simulink model "three_a_attitude_control_euler"  (R2021a)
settings: Solver=ode23t  StartTime=0.0  StopTime=100  RelTol=1e-5
undefined symbols (not defined in the file): eul_0, eul_init, g, I, km, kt, L, m, pm_0, sigbuilder_block, thrust_max, TQ_max_per_motor, Vb_init, Vm_0, wb_init, Xe_init, xme_0
libraries: simulink_extras x15, pid_lib x5, simulink x1
(part 1 of 2)
settings Model: Creator=Petronas-Tareq  LastModifiedBy=Petronas-Tareq

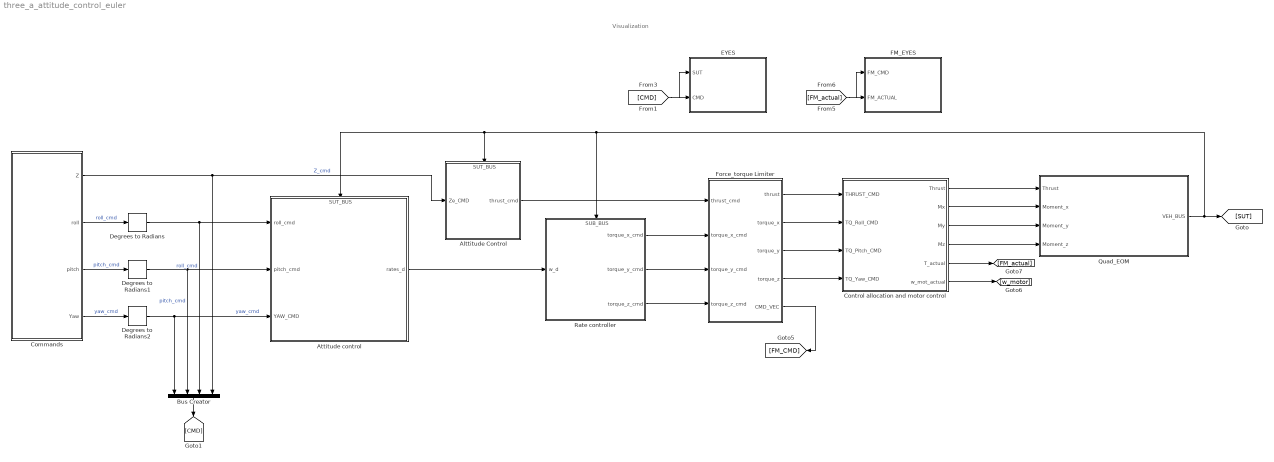
== system three_a_attitude_control_euler ==
  note: Visualization
  Alttitude Control : Subsystem
      settings: PortSchema="{\"entries\":[{\"content\":{\"sides\":[{\"content\":{\"connectorIds\":[\"In1\"]},\"type\":\"ConnectorPlacement.EquallySpacedRectSide\",\"uuid\":\"04a4dd9c-9e09-4d9f-8b40-74299d59d50a\"},{\"content\":{\"connectorIds\":[\"Out1\"],\"side\":\"RIGHT\"},\"type\":\"ConnectorPlacement.EquallySpacedRectSide\",\"uuid\":\"9fb2fefb-3382-44e9-a1a3-16b1599dcea5\"},{\"content\":{\"connectorIds\":[\"In2\"],\"side\":\"TOP\"},\"type\":\"ConnectorPlacement.EquallySpacedRectSide\",\"uuid\":\"ac10f64d-060e-4480-8a7d-828840fbd7d9\"}]},\"type\":\"ConnectorPlacement.EquallySpacedConnector\",\"uuid\":\"0b937044-8b2b-493f-9a2b-19b87fbfd9f1\"}],\"packageUris\":[\"http://schema.mathworks.com/mf0/Connector/R2020b\"],\"version\":\"1.0\"}"
  Attitude control : Subsystem
      settings: PortSchema="{\"entries\":[{\"content\":{\"sides\":[{\"content\":{\"connectorIds\":[\"In1\",\"In2\",\"In3\"]},\"type\":\"ConnectorPlacement.EquallySpacedRectSide\",\"uuid\":\"0f742873-dbcb-4fcb-ac41-98e78a79b9ee\"},{\"content\":{\"connectorIds\":[\"Out1\"],\"side\":\"RIGHT\"},\"type\":\"ConnectorPlacement.EquallySpacedRectSide\",\"uuid\":\"07146a16-46ee-4512-bd2a-6ffb0e678387\"},{\"content\":{\"connectorIds\":[\"In4\"],\"side\":\"TOP\"},\"type\":\"ConnectorPlacement.EquallySpacedRectSide\",\"uuid\":\"912b5acb-4e7e-41a0-b44d-ff207907913c\"}]},\"type\":\"ConnectorPlacement.EquallySpacedConnector\",\"uuid\":\"a7167a2e-3f96-46de-903f-90a596b85c06\"}],\"packageUris\":[\"http://schema.mathworks.com/mf0/Connector/R2020b\"],\"version\":\"1.0\"}"
      mask Display: image('$imagefile'); % Use "Edit Image" on toolstrip to change.
  Bus Creator : BusCreator  Inputs=4
  Commands : Subsystem  Variant=on  VariantControlMode=label  LabelModeActiveChoice=Choice_5
  Control allocation and motor control : Subsystem  Variant=on  VariantControlMode=label  LabelModeActiveChoice=Choice1
      mask Display: image('$imagefile'); % Use "Edit Image" on toolstrip to change.
  Degrees to Radians : simulink_extras/Transformations/Degrees to Radians
  Degrees to Radians1 : simulink_extras/Transformations/Degrees to Radians
  Degrees to Radians2 : simulink_extras/Transformations/Degrees to Radians
  EYES : Subsystem
  FM_EYES : Subsystem
  Force_torque Limiter : Subsystem
  Quad_EOM : Subsystem
      mask Display: image('$imagefile'); % Use "Edit Image" on toolstrip to change.
  Rate controller : Subsystem
      settings: PortSchema="{\"entries\":[{\"content\":{\"sides\":[{\"content\":{\"connectorIds\":[\"In1\"]},\"type\":\"ConnectorPlacement.EquallySpacedRectSide\",\"uuid\":\"0af60e35-7b10-4750-a6af-1a3d920b4771\"},{\"content\":{\"connectorIds\":[\"Out1\",\"Out2\",\"Out3\"],\"side\":\"RIGHT\"},\"type\":\"ConnectorPlacement.EquallySpacedRectSide\",\"uuid\":\"931b0f34-b3f1-4a41-949f-3d763eca3151\"},{\"content\":{\"connectorIds\":[\"In2\"],\"side\":\"TOP\"},\"type\":\"ConnectorPlacement.EquallySpacedRectSide\",\"uuid\":\"84fe42fa-07d1-4fd9-ad2f-8c6651eaa98c\"}]},\"type\":\"ConnectorPlacement.EquallySpacedConnector\",\"uuid\":\"f603d2ac-5c20-4a82-ba8b-1c7971d6778a\"}],\"packageUris\":[\"http://schema.mathworks.com/mf0/Connector/R2020b\"],\"version\":\"1.0\"}"
  wires:
  [FM_CMD] -> FM_EYES/1(FM_CMD)
  [FM_actual] -> FM_EYES/2(FM_ACTUAL)
  Commands/1(Z) -> Bus Creator/4, Alttitude Control/1(Ze_CMD)  "Z_cmd"
  Degrees to Radians/1 -> Attitude control/1(roll_cmd), Bus Creator/3  "roll_cmd"
  Degrees to Radians2/1 -> Attitude control/3(YAW_CMD), Bus Creator/1  "yaw_cmd"
  [SUT] -> EYES/1(SUT)
  [CMD] -> EYES/2(CMD)
  Bus Creator/1 -> [CMD]
  Degrees to Radians1/1 -> Attitude control/2(pitch_cmd), Bus Creator/2  "pitch_cmd"
  Commands/2(roll) -> Degrees to Radians/1  "roll_cmd"
  Commands/3(pitch) -> Degrees to Radians1/1  "pitch_cmd"
  Commands/4(Yaw) -> Degrees to Radians2/1  "yaw_cmd"
  Rate controller/1(torque_x_cmd) -> Force_torque Limiter/2(torque_x_cmd)
  Rate controller/2(torque_y_cmd) -> Force_torque Limiter/3(torque_y_cmd)
  Force_torque Limiter/4(torque_z) -> Control allocation and motor control/4(TQ_Yaw_CMD)
  Rate controller/3(torque_z_cmd) -> Force_torque Limiter/4(torque_z_cmd)
  Force_torque Limiter/1(thrust) -> Control allocation and motor control/1(THRUST_CMD)
  Force_torque Limiter/2(torque_x) -> Control allocation and motor control/2(TQ_Roll_CMD)
  Control allocation and motor control/3(My) -> Quad_EOM/3(Moment_y)
  Control allocation and motor control/2(Mx) -> Quad_EOM/2(Moment_x)
  Control allocation and motor control/6(w_mot_actual) -> [w_motor]
  Force_torque Limiter/3(torque_y) -> Control allocation and motor control/3(TQ_Pitch_CMD)
  Control allocation and motor control/4(Mz) -> Quad_EOM/4(Moment_z)
  Control allocation and motor control/1(Thrust) -> Quad_EOM/1(Thrust)
  Control allocation and motor control/5(T_actual) -> [FM_actual]
  Force_torque Limiter/5(CMD_VEC) -> [FM_CMD]
  Quad_EOM/1(VEH_BUS) -> Rate controller/2(SUB_BUS), Alttitude Control/2(SUT_BUS), Attitude control/4(SUT_BUS), [SUT]
  Alttitude Control/1(thrust_cmd) -> Force_torque Limiter/1(thrust_cmd)
  Attitude control/1(rates_d) -> Rate controller/1(w_d)

== system three_a_attitude_control_euler/Alttitude Control ==
  Ze_CMD : Inport
  SUT_BUS : Inport  Port=2
  Constant3 : Constant  Value=m
  Gain : Gain  Gain=-g
  Sum2 : Sum  Inputs=++|
  Z_CONT1 : Subsystem
  thrust_cmd : Outport
  wires:
  Z_CONT1/1(THRUST) -> Sum2/2
  Constant3/1 -> Gain/1
  SUT_BUS/1 -> Z_CONT1/2(SUT_BUS)
  Gain/1 -> Sum2/1
  Ze_CMD/1 -> Z_CONT1/1(Ze_CMD)
  Sum2/1 -> thrust_cmd/1

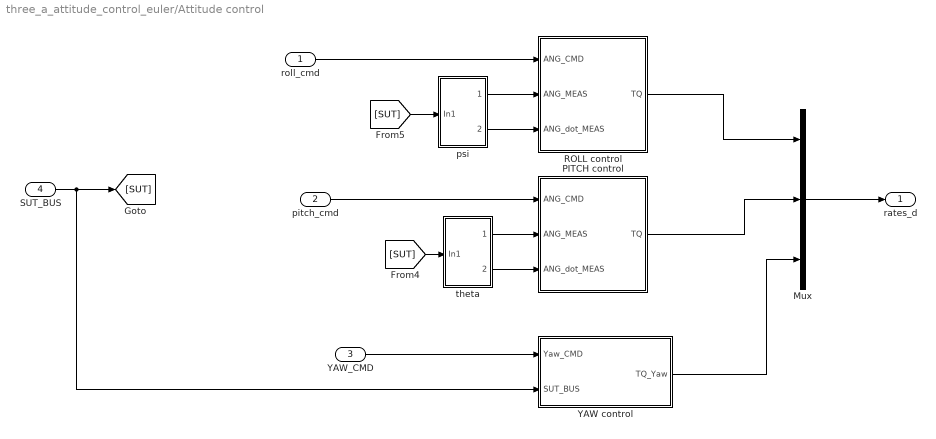
== system three_a_attitude_control_euler/Attitude control ==
  roll_cmd : Inport
  pitch_cmd : Inport  Port=2
  YAW_CMD : Inport  Port=3
  SUT_BUS : Inport  Port=4
  Mux : Mux  Inputs=3
  PITCH control : Subsystem
  ROLL control : Subsystem
  YAW control : Subsystem
  psi : Subsystem
  theta : Subsystem
  rates_d : Outport
  wires:
  SUT_BUS/1 -> [SUT], YAW control/2(SUT_BUS)
  YAW_CMD/1 -> YAW control/1(Yaw_CMD)
  [SUT] -> psi/1(In1)
  psi/2(Out2) -> ROLL control/3(ANG_dot_MEAS)
  psi/1(ANG_MEAS) -> ROLL control/2(ANG_MEAS)
  [SUT] -> theta/1(In1)
  theta/1(ANG_MEAS) -> PITCH control/2(ANG_MEAS)
  theta/2(ANG_dot_MEAS) -> PITCH control/3(ANG_dot_MEAS)
  pitch_cmd/1 -> PITCH control/1(ANG_CMD)
  roll_cmd/1 -> ROLL control/1(ANG_CMD)
  ROLL control/1(TQ) -> Mux/1
  PITCH control/1(TQ) -> Mux/2
  YAW control/1(TQ_Yaw) -> Mux/3
  Mux/1 -> rates_d/1

== system three_a_attitude_control_euler/Commands ==
  note: 1) Add Subsystem or Model blocks as valid variant choices.
      | 2) You cannot connect blocks at this level. At simulation, connectivity is automatically
      | determined, based on the active variant and port name matching.
  Acro : Subsystem  Tag=STV Subsys  LoadFcn=sigbuilder_block('load');  StartFcn=sigbuilder_block('start');  StopFcn=sigbuilder_block('stop');  ClipboardFcn=sigbuilder_block('clipboard');  VariantControl=Choice_6  mask(Sigbuilder block){tuvar=[0:10]}
      mask help: Simulink:masks:SigbuilderBlock_MD
      mask init:
      | if ~strcmp(get_param(bdroot(gcbh),'SimulationStatus'),'stopped') tuvar = sigbuilder_block('maskInit'); end
      settings: CopyFcn=sigbuilder_block('copy');  DeleteFcn=sigbuilder_block('delete');  ModelCloseFcn=sigbuilder_block('modelClose');  PreSaveFcn=sigbuilder_block('preSave');  PauseFcn=sigbuilder_block('pause');  ContinueFcn=sigbuilder_block('continue');  NameChangeFcn=sigbuilder_block('namechange');  OpenFcn=sigbuilder_block('open',[200.1 155.1 551.4 400.5 ]);  CloseFcn=sigbuilder_block('close');
      mask Display: plot(0, 0, 100, 100,[2, 2, 32, 32, 2], [68, 8, 8, 68, 68],[32, 2], [38, 38], [32, 19, 2],[53, 60, 44], [32, 17, 17, 2],[16, 16, 31, 31]);txt = getActiveGroup(gcbh);text(2, 100, txt,'verticalAlignment', 'top');
  "Altitude " : Subsystem  Tag=STV Subsys  LoadFcn=sigbuilder_block('load');  StartFcn=sigbuilder_block('start');  StopFcn=sigbuilder_block('stop');  ClipboardFcn=sigbuilder_block('clipboard');  VariantControl=Choice_1  mask(Sigbuilder block){tuvar=[0:10]}
      mask help: Simulink:masks:SigbuilderBlock_MD
      mask init:
      | if ~strcmp(get_param(bdroot(gcbh),'SimulationStatus'),'stopped') tuvar = sigbuilder_block('maskInit'); end
      settings: CopyFcn=sigbuilder_block('copy');  DeleteFcn=sigbuilder_block('delete');  ModelCloseFcn=sigbuilder_block('modelClose');  PreSaveFcn=sigbuilder_block('preSave');  PauseFcn=sigbuilder_block('pause');  ContinueFcn=sigbuilder_block('continue');  NameChangeFcn=sigbuilder_block('namechange');  OpenFcn=sigbuilder_block('open',[200.1 155.1 551.4 400.5 ]);  CloseFcn=sigbuilder_block('close');
      mask Display: plot(0, 0, 100, 100,[2, 2, 32, 32, 2], [68, 8, 8, 68, 68],[32, 2], [38, 38], [32, 19, 2],[53, 60, 44], [32, 17, 17, 2],[16, 16, 31, 31]);txt = getActiveGroup(gcbh);text(2, 100, txt,'verticalAlignment', 'top');
  Ground : Subsystem  Tag=STV Subsys  LoadFcn=sigbuilder_block('load');  StartFcn=sigbuilder_block('start');  StopFcn=sigbuilder_block('stop');  ClipboardFcn=sigbuilder_block('clipboard');  VariantControl=Choice  mask(Sigbuilder block){tuvar=[0:10]}
      mask help: Simulink:masks:SigbuilderBlock_MD
      mask init:
      | if ~strcmp(get_param(bdroot(gcbh),'SimulationStatus'),'stopped') tuvar = sigbuilder_block('maskInit'); end
      settings: CopyFcn=sigbuilder_block('copy');  DeleteFcn=sigbuilder_block('delete');  ModelCloseFcn=sigbuilder_block('modelClose');  PreSaveFcn=sigbuilder_block('preSave');  PauseFcn=sigbuilder_block('pause');  ContinueFcn=sigbuilder_block('continue');  NameChangeFcn=sigbuilder_block('namechange');  OpenFcn=sigbuilder_block('open',[200.1 155.1 551.4 400.5 ]);  CloseFcn=sigbuilder_block('close');
      mask Display: plot(0, 0, 100, 100,[2, 2, 32, 32, 2], [68, 8, 8, 68, 68],[32, 2], [38, 38], [32, 19, 2],[53, 60, 44], [32, 17, 17, 2],[16, 16, 31, 31]);txt = getActiveGroup(gcbh);text(2, 100, txt,'verticalAlignment', 'top');
  Pitch : Subsystem  Tag=STV Subsys  LoadFcn=sigbuilder_block('load');  StartFcn=sigbuilder_block('start');  StopFcn=sigbuilder_block('stop');  ClipboardFcn=sigbuilder_block('clipboard');  VariantControl=Choice_3  mask(Sigbuilder block){tuvar=[0:10]}
      mask help: Simulink:masks:SigbuilderBlock_MD
      mask init:
      | if ~strcmp(get_param(bdroot(gcbh),'SimulationStatus'),'stopped') tuvar = sigbuilder_block('maskInit'); end
      settings: CopyFcn=sigbuilder_block('copy');  DeleteFcn=sigbuilder_block('delete');  ModelCloseFcn=sigbuilder_block('modelClose');  PreSaveFcn=sigbuilder_block('preSave');  PauseFcn=sigbuilder_block('pause');  ContinueFcn=sigbuilder_block('continue');  NameChangeFcn=sigbuilder_block('namechange');  OpenFcn=sigbuilder_block('open',[452.4 149.7 551.4 400.5 ]);  CloseFcn=sigbuilder_block('close');
      mask Display: plot(0, 0, 100, 100,[2, 2, 32, 32, 2], [68, 8, 8, 68, 68],[32, 2], [38, 38], [32, 19, 2],[53, 60, 44], [32, 17, 17, 2],[16, 16, 31, 31]);txt = getActiveGroup(gcbh);text(2, 100, txt,'verticalAlignment', 'top');
  Roll : Subsystem  Tag=STV Subsys  LoadFcn=sigbuilder_block('load');  StartFcn=sigbuilder_block('start');  StopFcn=sigbuilder_block('stop');  ClipboardFcn=sigbuilder_block('clipboard');  VariantControl=Choice_2  mask(Sigbuilder block){tuvar=[0:10]}
      mask help: Simulink:masks:SigbuilderBlock_MD
      mask init:
      | if ~strcmp(get_param(bdroot(gcbh),'SimulationStatus'),'stopped') tuvar = sigbuilder_block('maskInit'); end
      settings: CopyFcn=sigbuilder_block('copy');  DeleteFcn=sigbuilder_block('delete');  ModelCloseFcn=sigbuilder_block('modelClose');  PreSaveFcn=sigbuilder_block('preSave');  PauseFcn=sigbuilder_block('pause');  ContinueFcn=sigbuilder_block('continue');  NameChangeFcn=sigbuilder_block('namechange');  OpenFcn=sigbuilder_block('open',[452.4 149.7 551.4 400.5 ]);  CloseFcn=sigbuilder_block('close');
      mask Display: plot(0, 0, 100, 100,[2, 2, 32, 32, 2], [68, 8, 8, 68, 68],[32, 2], [38, 38], [32, 19, 2],[53, 60, 44], [32, 17, 17, 2],[16, 16, 31, 31]);txt = getActiveGroup(gcbh);text(2, 100, txt,'verticalAlignment', 'top');
  multisteps : Subsystem  Tag=STV Subsys  LoadFcn=sigbuilder_block('load');  StartFcn=sigbuilder_block('start');  StopFcn=sigbuilder_block('stop');  ClipboardFcn=sigbuilder_block('clipboard');  VariantControl=Choice_5  mask(Sigbuilder block){tuvar=[0:10]}
      mask help: Simulink:masks:SigbuilderBlock_MD
      mask init:
      | if ~strcmp(get_param(bdroot(gcbh),'SimulationStatus'),'stopped') tuvar = sigbuilder_block('maskInit'); end
      settings: CopyFcn=sigbuilder_block('copy');  DeleteFcn=sigbuilder_block('delete');  ModelCloseFcn=sigbuilder_block('modelClose');  PreSaveFcn=sigbuilder_block('preSave');  PauseFcn=sigbuilder_block('pause');  ContinueFcn=sigbuilder_block('continue');  NameChangeFcn=sigbuilder_block('namechange');  OpenFcn=sigbuilder_block('open',[200.1 155.1 551.4 400.5 ]);  CloseFcn=sigbuilder_block('close');
      mask Display: plot(0, 0, 100, 100,[2, 2, 32, 32, 2], [68, 8, 8, 68, 68],[32, 2], [38, 38], [32, 19, 2],[53, 60, 44], [32, 17, 17, 2],[16, 16, 31, 31]);txt = getActiveGroup(gcbh);text(2, 100, txt,'verticalAlignment', 'top');
  yaw : Subsystem  Tag=STV Subsys  LoadFcn=sigbuilder_block('load');  StartFcn=sigbuilder_block('start');  StopFcn=sigbuilder_block('stop');  ClipboardFcn=sigbuilder_block('clipboard');  VariantControl=Choice_4  mask(Sigbuilder block){tuvar=[0:10]}
      mask help: Simulink:masks:SigbuilderBlock_MD
      mask init:
      | if ~strcmp(get_param(bdroot(gcbh),'SimulationStatus'),'stopped') tuvar = sigbuilder_block('maskInit'); end
      settings: CopyFcn=sigbuilder_block('copy');  DeleteFcn=sigbuilder_block('delete');  ModelCloseFcn=sigbuilder_block('modelClose');  PreSaveFcn=sigbuilder_block('preSave');  PauseFcn=sigbuilder_block('pause');  ContinueFcn=sigbuilder_block('continue');  NameChangeFcn=sigbuilder_block('namechange');  OpenFcn=sigbuilder_block('open',[452.4 149.7 551.4 400.5 ]);  CloseFcn=sigbuilder_block('close');
      mask Display: plot(0, 0, 100, 100,[2, 2, 32, 32, 2], [68, 8, 8, 68, 68],[32, 2], [38, 38], [32, 19, 2],[53, 60, 44], [32, 17, 17, 2],[16, 16, 31, 31]);txt = getActiveGroup(gcbh);text(2, 100, txt,'verticalAlignment', 'top');
  Z : Outport
  roll : Outport  Port=2
  pitch : Outport  Port=3
  Yaw : Outport  Port=4

== system three_a_attitude_control_euler/Control allocation and motor control ==
  note: 1) Add Subsystem or Model blocks as valid variant choices.
      | 2) You cannot connect blocks at this level. At simulation, connectivity is automatically
      | determined, based on the active variant and port name matching.
  THRUST_CMD : Inport
  TQ_Roll_CMD : Inport  Port=2
  TQ_Pitch_CMD : Inport  Port=3
  TQ_Yaw_CMD : Inport  Port=4
  Ideal Actuators with allocation : Subsystem  VariantControl=Choice2
  Ideal Actuattion (direct transfer) : Subsystem  VariantControl=Choice1
  Thrust : Outport
  Mx : Outport  Port=2
  My : Outport  Port=3
  Mz : Outport  Port=4
  T_actual : Outport  Port=5
  w_mot_actual : Outport  Port=6

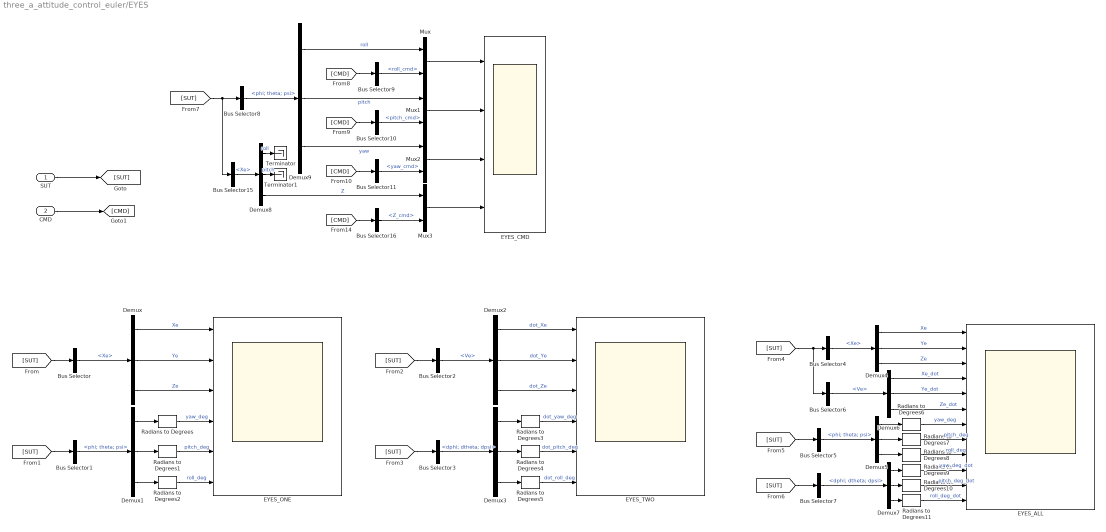
== system three_a_attitude_control_euler/EYES ==
  SUT : Inport
  CMD : Inport  Port=2
  Bus Selector : BusSelector  OutputSignals=Xe
  Bus Selector1 : BusSelector  OutputSignals=phi; theta; psi
  Bus Selector10 : BusSelector  OutputSignals=pitch_cmd
  Bus Selector11 : BusSelector  OutputSignals=yaw_cmd
  Bus Selector15 : BusSelector  OutputSignals=Xe
  Bus Selector16 : BusSelector  OutputSignals=Z_cmd
  Bus Selector2 : BusSelector  OutputSignals=Ve
  Bus Selector3 : BusSelector  OutputSignals=dphi; dtheta; dpsi
  Bus Selector4 : BusSelector  OutputSignals=Xe
  Bus Selector5 : BusSelector  OutputSignals=phi; theta; psi
  Bus Selector6 : BusSelector  OutputSignals=Ve
  Bus Selector7 : BusSelector  OutputSignals=dphi; dtheta; dpsi
  Bus Selector8 : BusSelector  OutputSignals=phi; theta; psi
  Bus Selector9 : BusSelector  OutputSignals=roll_cmd
  Demux{,1..9} (10 alike) : Demux  Outputs=3
  EYES_ALL : Scope  NumInputPorts=12
  EYES_CMD : Scope  NumInputPorts=4
  EYES_ONE : Scope  NumInputPorts=6
  EYES_TWO : Scope  NumInputPorts=6
  Mux{,1..3} (4 alike) : Mux  Inputs=2
  Radians to Degrees{,1..11} (12 alike) : simulink_extras/Transformations/Radians to Degrees
  Terminator : Terminator
  Terminator1 : Terminator
  wires:
  SUT/1 -> [SUT]
  [SUT] -> Bus Selector/1
  Demux/2 -> EYES_ONE/2  "Ye"
  Demux/3 -> EYES_ONE/3  "Ze"
  Demux/1 -> EYES_ONE/1  "Xe"
  Bus Selector/1 -> Demux/1  "<Xe>"
  Bus Selector1/1 -> Demux1/1  "<phi; theta; psi>"
  [SUT] -> Bus Selector1/1
  Demux1/1 -> Radians to Degrees/1
  Radians to Degrees/1 -> EYES_ONE/4  "yaw_deg"
  Radians to Degrees1/1 -> EYES_ONE/5  "pitch_deg"
  Radians to Degrees2/1 -> EYES_ONE/6  "roll_deg"
  Demux1/3 -> Radians to Degrees2/1
  Demux1/2 -> Radians to Degrees1/1
  [SUT] -> Bus Selector2/1
  Demux2/2 -> EYES_TWO/2  "dot_Ye"
  Demux2/3 -> EYES_TWO/3  "dot_Ze"
  Demux2/1 -> EYES_TWO/1  "dot_Xe"
  Bus Selector2/1 -> Demux2/1  "<Ve>"
  Bus Selector3/1 -> Demux3/1  "<dphi; dtheta; dpsi>"
  [SUT] -> Bus Selector3/1
  Demux3/1 -> Radians to Degrees3/1
  Radians to Degrees3/1 -> EYES_TWO/4  "dot_yaw_deg"
  Radians to Degrees4/1 -> EYES_TWO/5  "dot_pitch_deg"
  Radians to Degrees5/1 -> EYES_TWO/6  "dot_roll_deg"
  Demux3/3 -> Radians to Degrees5/1
  Demux3/2 -> Radians to Degrees4/1
  [SUT] -> Bus Selector6/1, Bus Selector4/1
  Demux4/2 -> EYES_ALL/2  "Ye"
  Demux4/3 -> EYES_ALL/3  "Ze"
  Demux4/1 -> EYES_ALL/1  "Xe"
  Bus Selector4/1 -> Demux4/1  "<Xe>"
  Bus Selector5/1 -> Demux5/1  "<phi; theta; psi>"
  [SUT] -> Bus Selector5/1
  Demux5/1 -> Radians to Degrees6/1
  Demux6/1 -> EYES_ALL/4  "Xe_dot"
  Demux6/2 -> EYES_ALL/5  "Ye_dot"
  Demux6/3 -> EYES_ALL/6  "Ze_dot"
  Demux5/3 -> Radians to Degrees8/1
  Demux5/2 -> Radians to Degrees7/1
  Bus Selector6/1 -> Demux6/1  "<Ve>"
  Radians to Degrees6/1 -> EYES_ALL/7  "yaw_deg"
  Radians to Degrees7/1 -> EYES_ALL/8  "pitch_deg"
  Radians to Degrees8/1 -> EYES_ALL/9  "roll_deg"
  Bus Selector7/1 -> Demux7/1  "<dphi; dtheta; dpsi>"
  [SUT] -> Bus Selector7/1
  Demux7/1 -> Radians to Degrees9/1
  Demux7/2 -> Radians to Degrees10/1
  Demux7/3 -> Radians to Degrees11/1
  Radians to Degrees9/1 -> EYES_ALL/10  "yaw_deg_dot"
  Radians to Degrees10/1 -> EYES_ALL/11  "pitch_deg_dot"
  Radians to Degrees11/1 -> EYES_ALL/12  "roll_deg_dot"
  CMD/1 -> [CMD]
  [SUT] -> Bus Selector8/1, Bus Selector15/1
  Demux9/2 -> Mux1/1  "pitch"
  Demux9/1 -> Mux/1  "roll"
  Bus Selector8/1 -> Demux9/1  "<phi; theta; psi>"
  Mux/1 -> EYES_CMD/1
  Mux1/1 -> EYES_CMD/2
  Mux2/1 -> EYES_CMD/3
  Demux9/3 -> Mux2/1  "yaw"
  [CMD] -> Bus Selector9/1
  Bus Selector9/1 -> Mux/2  "<roll_cmd>"
  [CMD] -> Bus Selector10/1
  Bus Selector10/1 -> Mux1/2  "<pitch_cmd>"
  [CMD] -> Bus Selector11/1
  Bus Selector11/1 -> Mux2/2  "<yaw_cmd>"
  Bus Selector15/1 -> Demux8/1  "<Xe>"
  Demux8/1 -> Terminator/1  "roll"
  Demux8/2 -> Terminator1/1  "pitch"
  Bus Selector16/1 -> Mux3/2  "<Z_cmd>"
  [CMD] -> Bus Selector16/1
  Mux3/1 -> EYES_CMD/4
  Demux8/3 -> Mux3/1  "Z"

== system three_a_attitude_control_euler/FM_EYES ==
  FM_CMD : Inport
  FM_ACTUAL : Inport  Port=2
  FM CMD vs Actual : Scope  NumInputPorts=4
  FM_Mux : Subsystem
  wires:
  FM_CMD/1 -> [FM_CMD]
  [FM_CMD] -> FM_Mux/1(FM_CMD)
  [FM] -> FM_Mux/2(FM)
  FM_Mux/1(Y1) -> FM CMD vs Actual/1  "Thrust"
  FM_Mux/2(Y2) -> FM CMD vs Actual/2  "TQ_Roll_X"
  FM_Mux/3(w3) -> FM CMD vs Actual/3  "TQ_Pitch_Y"
  FM_Mux/4(Y4) -> FM CMD vs Actual/4  "TQ_Yaw_Z"
  FM_ACTUAL/1 -> [FM]

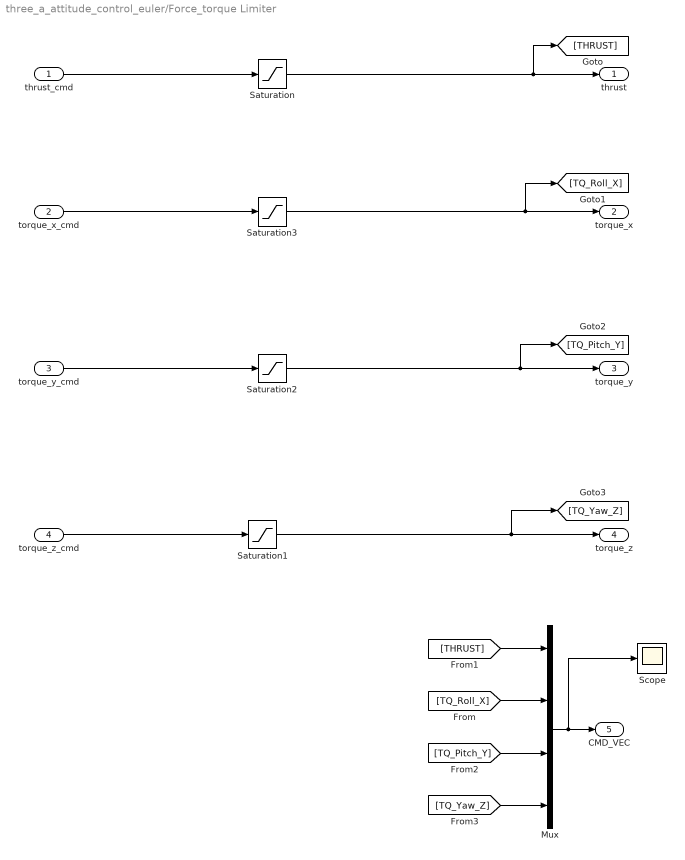
== system three_a_attitude_control_euler/Force_torque Limiter ==
  thrust_cmd : Inport
  torque_x_cmd : Inport  Port=2
  torque_y_cmd : Inport  Port=3
  torque_z_cmd : Inport  Port=4
  Mux : Mux
  Saturation : Saturate  UpperLimit=4*thrust_max  LowerLimit=-4*thrust_max
      settings: AttributesFormatString=|
      | MAX =    %<UpperLimit>
      | MIN = %<LowerLimit>
  Saturation1 : Saturate  UpperLimit=2*TQ_max_per_motor  LowerLimit=-2*TQ_max_per_motor
      settings: AttributesFormatString=|
      | MAX =    %<UpperLimit>
      | MIN = %<LowerLimit>
  Saturation2 : Saturate  UpperLimit="thrust_max *  L"  LowerLimit=-thrust_max *L
      settings: AttributesFormatString=|
      | MAX =    %<UpperLimit>
      | MIN = %<LowerLimit>
  Saturation3 : Saturate  UpperLimit=thrust_max *L  LowerLimit=-thrust_max *L
      settings: AttributesFormatString=|
      | MAX =    %<UpperLimit>
      | MIN = %<LowerLimit>
  Scope : Scope
  thrust : Outport  VectorParamsAs1DForOutWhenUnconnected=off
  torque_x : Outport  Port=2  VectorParamsAs1DForOutWhenUnconnected=off
  torque_y : Outport  Port=3  VectorParamsAs1DForOutWhenUnconnected=off
  torque_z : Outport  Port=4  VectorParamsAs1DForOutWhenUnconnected=off
  CMD_VEC : Outport  Port=5  VectorParamsAs1DForOutWhenUnconnected=off
  wires:
  torque_z_cmd/1 -> Saturation1/1
  thrust_cmd/1 -> Saturation/1
  torque_y_cmd/1 -> Saturation2/1
  torque_x_cmd/1 -> Saturation3/1
  Saturation/1 -> [THRUST], thrust/1
  Saturation3/1 -> [TQ_Roll_X], torque_x/1
  Saturation2/1 -> [TQ_Pitch_Y], torque_y/1
  Saturation1/1 -> [TQ_Yaw_Z], torque_z/1
  Mux/1 -> Scope/1, CMD_VEC/1
  [THRUST] -> Mux/1
  [TQ_Roll_X] -> Mux/2
  [TQ_Pitch_Y] -> Mux/3
  [TQ_Yaw_Z] -> Mux/4

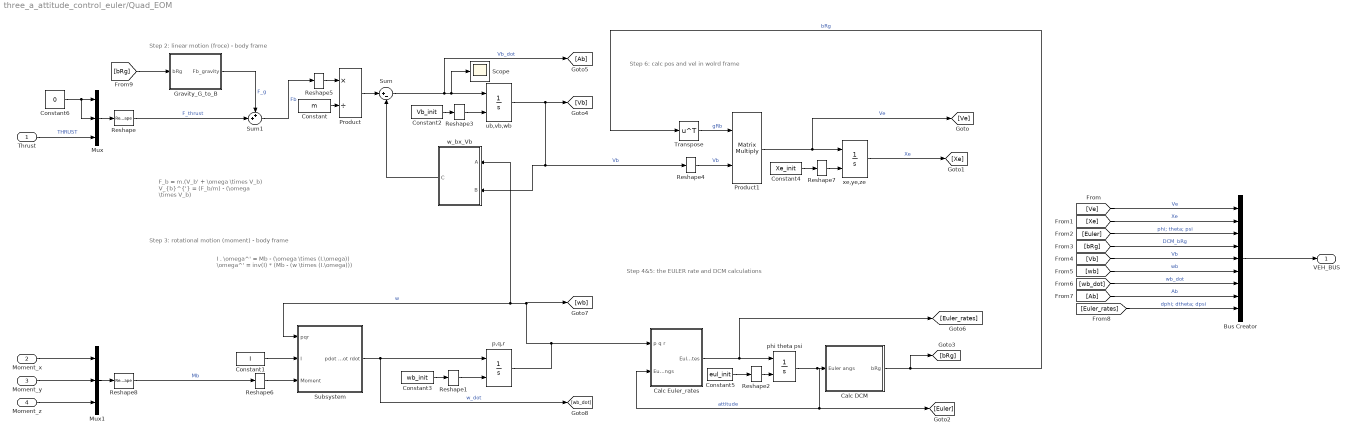
== system three_a_attitude_control_euler/Quad_EOM ==
  note: Step 3: rotational motion (moment) - body frame
  note: F_b = m.(V_b' + \omega \times V_b)
      |
      | V_{b}^{'} = (F_b/m) - (\omega \times V_b)
  note: Step 2: linear motion (froce) - body frame
  note: Step 6: calc pos and vel in wolrd frame
  note: I . \omega^' = Mb - (\omega \times (I.\omega))
      |
      | \omega^' = inv(I) * (Mb - (w \times (I.\omega)))
  note: Step 4&5: the EULER rate and DCM calculations
  Thrust : Inport
  Moment_x : Inport  Port=2
  Moment_y : Inport  Port=3
  Moment_z : Inport  Port=4
  Bus Creator : BusCreator  Inputs=9
  Calc DCM : Subsystem
  Calc Euler_rates : Subsystem
  Constant : Constant  Value=m  OutDataTypeStr=Inherit: Inherit via back propagation
  Constant1 : Constant  Value=I  OutDataTypeStr=Inherit: Inherit via back propagation
  Constant2 : Constant  Value=Vb_init  OutDataTypeStr=Inherit: Inherit via back propagation
  Constant3 : Constant  Value=wb_init  OutDataTypeStr=Inherit: Inherit via back propagation
  Constant4 : Constant  Value=Xe_init  OutDataTypeStr=Inherit: Inherit via back propagation
  Constant5 : Constant  Value=eul_init  OutDataTypeStr=Inherit: Inherit via back propagation
  Constant6 : Constant  Value=0
  Gravity_G_to_B : Subsystem
  Mux : Mux  Inputs=3
  Mux1 : Mux  Inputs=3
  Product : Product  Inputs=*/  SaturateOnIntegerOverflow=on  OutDataTypeStr=Inherit: Same as first input
  Product1 : Product  Multiplication=Matrix(*)  InputSameDT=on  SaturateOnIntegerOverflow=on  OutDataTypeStr=Inherit: Same as first input
  Reshape{,1..8} (9 alike) : Reshape  OutputDimensionality=Column vector (2-D)
  Scope : Scope
  Subsystem : Subsystem
  Sum : Sum  Inputs=|+-  SaturateOnIntegerOverflow=on
  Sum1 : Sum  Inputs=++|
  Transpose : Math  Operator=transpose  SignedPower=on  SaturateOnIntegerOverflow=on
  "p,q,r " : Integrator  InitialConditionSource=external  InitialCondition=pm_0
  phi theta psi : Integrator  InitialConditionSource=external  InitialCondition=eul_0
  ub,vb,wb : Integrator  InitialConditionSource=external  InitialCondition=Vm_0
  w_bx_Vb : Subsystem
      mask Display:
      | text(.5,.5,'Cross\nProduct\n\nC = AxB', ...
      | 	'HorizontalAlignment','Center',...
      | 	'VerticalAlignment','middle')
  xe,ye,ze : Integrator  InitialConditionSource=external  InitialCondition=xme_0
  VEH_BUS : Outport  VectorParamsAs1DForOutWhenUnconnected=off
  wires:
  [Euler] -> Bus Creator/3  "phi; theta; psi"
  [Xe] -> Bus Creator/2  "Xe"
  [Ve] -> Bus Creator/1  "Ve"
  [bRg] -> Bus Creator/4  "DCM_bRg"
  [Ab] -> Bus Creator/8  "Ab"
  [wb_dot] -> Bus Creator/7  "wb_dot"
  Bus Creator/1 -> VEH_BUS/1
  [Vb] -> Bus Creator/5  "Vb"
  [wb] -> Bus Creator/6  "wb"
  [Euler_rates] -> Bus Creator/9  "dphi; dtheta; dpsi"
  Reshape8/1 -> Reshape6/1  "Mb"
  Reshape6/1 -> Subsystem/3(Moment)
  Constant5/1 -> Reshape2/1
  Reshape1/1 -> "p,q,r "/2
  Transpose/1 -> Product1/1  "gRb"
  Constant2/1 -> Reshape3/1
  Subsystem/1(pdot qdot rdot) -> [wb_dot], "p,q,r "/1  "w_dot"
  Constant/1 -> Product/2
  Constant1/1 -> Subsystem/2(I)
  Reshape4/1 -> Product1/2  "Vb"
  w_bx_Vb/1(C) -> Sum/2
  Calc DCM/1(bRg) -> [bRg], Transpose/1  "bRg"
  Calc Euler_rates/1(Euler_rates) -> [Euler_rates], phi theta psi/1
  Reshape2/1 -> phi theta psi/2
  Sum/1 -> [Ab], Scope/1, ub,vb,wb/1  "Vb_dot"
  Constant4/1 -> Reshape7/1
  Reshape3/1 -> ub,vb,wb/2
  Reshape7/1 -> xe,ye,ze/2
  Product1/1 -> [Ve], xe,ye,ze/1  "Ve"
  Reshape5/1 -> Product/1
  xe,ye,ze/1 -> [Xe]  "Xe"
  Sum1/1 -> Reshape5/1  "Fb"
  Constant3/1 -> Reshape1/1
  Product/1 -> Sum/1
  Constant6/1 -> Mux/2, Mux/1
  Gravity_G_to_B/1(Fb_gravity) -> Sum1/1  "F_g"
  Mux/1 -> Reshape/1
  Reshape/1 -> Sum1/2  "F_thrust"
  Thrust/1 -> Mux/3  "THRUST"
  [bRg] -> Gravity_G_to_B/1(bRg)
  Moment_y/1 -> Mux1/2
  Moment_z/1 -> Mux1/3
  Mux1/1 -> Reshape8/1
  Moment_x/1 -> Mux1/1
  "p,q,r "/1 -> [wb], Subsystem/1(pqr), w_bx_Vb/1(A), Calc Euler_rates/1("p q r ")  "w"
  ub,vb,wb/1 -> [Vb], w_bx_Vb/2(B), Reshape4/1  "Vb"
  phi theta psi/1 -> Calc DCM/1(Euler angs), Calc Euler_rates/2(Euler_angs), [Euler]  "attitude"

== system three_a_attitude_control_euler/Rate controller ==
  note: Rate controller
  w_d : Inport
  SUB_BUS : Inport  Port=2
  Bus Selector1 : BusSelector  OutputSignals=wb,wb_dot
  Demux : Demux  Outputs=3
  Kd_rates : Gain  Gain=0.1
  Kp_rates : Gain  Gain=5
  Scope : Scope  NumInputPorts=2
  Sum : Sum  Inputs=|+-
  Sum1 : Sum  Inputs=|+-
  torque_x_cmd : Outport
  torque_y_cmd : Outport  Port=2
  torque_z_cmd : Outport  Port=3
  wires:
  Bus Selector1/2 -> Kd_rates/1  "<wb_dot>"
  Bus Selector1/1 -> Sum1/2, Scope/2  "<wb>"
  Demux/1 -> torque_x_cmd/1
  Demux/2 -> torque_y_cmd/1
  Demux/3 -> torque_z_cmd/1
  SUB_BUS/1 -> Bus Selector1/1  "measurements"
  w_d/1 -> Sum1/1, Scope/1
  Kd_rates/1 -> Sum/2  "w_d"
  Kp_rates/1 -> Sum/1
  Sum/1 -> Demux/1  "torques"
  Sum1/1 -> Kp_rates/1

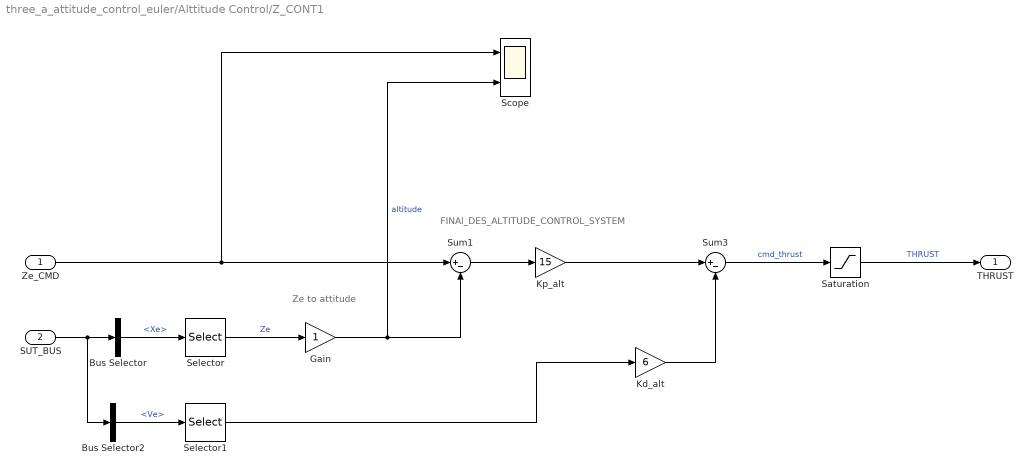
== system three_a_attitude_control_euler/Alttitude Control/Z_CONT1 ==
  note: FINAl_DES_ALTITUDE_CONTROL_SYSTEM
  note: Ze to attitude
  Ze_CMD : Inport
  SUT_BUS : Inport  Port=2
  Bus Selector : BusSelector  OutputSignals=Xe
  Bus Selector2 : BusSelector  OutputSignals=Ve
  Gain : Gain
  Kd_alt : Gain  Gain=6
  Kp_alt : Gain  Gain=15
  Saturation : Saturate  UpperLimit=4*thrust_max  LowerLimit=-4*thrust_max
  Scope : Scope  NumInputPorts=2
  Selector : Selector  InputPortWidth=3  IndexOptions=Index vector (dialog)  Indices=3  OutputSizes=1
  Selector1 : Selector  InputPortWidth=3  IndexOptions=Index vector (dialog)  Indices=3  OutputSizes=1
  Sum1 : Sum  Inputs=|+-
  Sum3 : Sum  Inputs=|+-
  THRUST : Outport  VectorParamsAs1DForOutWhenUnconnected=off
  wires:
  Gain/1 -> Sum1/2, Scope/2  "altitude"
  SUT_BUS/1 -> Bus Selector2/1, Bus Selector/1
  Bus Selector2/1 -> Selector1/1  "<Ve>"
  Bus Selector/1 -> Selector/1  "<Xe>"
  Selector/1 -> Gain/1  "Ze"
  Kd_alt/1 -> Sum3/2
  Selector1/1 -> Kd_alt/1
  Kp_alt/1 -> Sum3/1
  Saturation/1 -> THRUST/1  "THRUST"
  Sum3/1 -> Saturation/1  "cmd_thrust"
  Ze_CMD/1 -> Sum1/1, Scope/1
  Sum1/1 -> Kp_alt/1

== system three_a_attitude_control_euler/Attitude control/PITCH control ==
  note: NOTE: 1 radian = 57 degrees
  ANG_CMD : Inport
  ANG_MEAS : Inport  Port=2
  ANG_dot_MEAS : Inport  Port=3
  P_CONT : pid_lib/PID Controller  Controller=P  Form=Parallel  TimeDomain=Continuous-time  UseExternalTs=off  SampleTime=-1  IntegratorMethod=Forward Euler  FilterMethod=Forward Euler  ControllerParametersSource=internal  P=1  I=7.09690484808648  D=-0.334898279224841  UseFilter=on  N=17.076664592689  TunerSelectOption=Transfer Function Based (PID Tuner App)  InitialConditionSource=internal  InitialConditionForIntegrator=0  InitialConditionForFilter=0  DifferentiatorICPrevScaledInput=0  ExternalReset=none  TrackingMode=off  Kt=1  LimitOutput=off  SatLimitsSource=internal  UpperSaturationLimit=inf  LowerSaturationLimit=-inf  LinearizeAsGain=on  AntiWindupMode=none  Kb=1  POutMin=[]  POutMax=[]  IOutMin=[]  IOutMax=[]  DOutMin=[]  DOutMax=[]  NOutMin=[]  NOutMax=[]  SumOutMin=[]  SumOutMax=[]  SaturationOutMin=[]  SaturationOutMax=[]  PParamMin=[]  PParamMax=[]  IParamMin=[]  IParamMax=[]  DParamMin=[]  DParamMax=[]  NParamMin=[]  NParamMax=[]  KbParamMin=[]  KbParamMax=[]  KtParamMin=[]  KtParamMax=[]  KbOutMin=[]  KbOutMax=[]  KtOutMin=[]  KtOutMax=[]  IntegratorOutMin=[]  IntegratorOutMax=[]  FilterOutMin=[]  FilterOutMax=[]  SumI1OutMin=[]  SumI1OutMax=[]  SumI2OutMin=[]  SumI2OutMax=[]  SumI3OutMin=[]  SumI3OutMax=[]  SumI4OutMin=[]  SumI4OutMax=[]  SumDOutMin=[]  SumDOutMax=[]  DifferentiatorOutMin=[]  DifferentiatorOutMax=[]  FilterDiffOutCoefMin=[]  FilterDiffOutCoefMax=[]  ReciprocalOutMin=[]  ReciprocalOutMax=[]  SumDenOutMin=[]  SumDenOutMax=[]  SumNumOutMin=[]  SumNumOutMax=[]  DivideOutMin=[]  DivideOutMax=[]  UdiffTsProdOutMin=[]  UdiffTsProdOutMax=[]  NTsProdOutMin=[]  NTsProdOutMax=[]  UintegralTsProdOutMin=[]  UintegralTsProdOutMax=[]  UngainTsProdOutMin=[]  UngainTsProdOutMax=[]  IntegratorContinuousStateAttributes=''  IntegratorStateMustResolveToSignalObject=off  IntegratorRTWStateStorageClass=Auto  FilterContinuousStateAttributes=''  FilterStateMustResolveToSignalObject=off  FilterRTWStateStorageClass=Auto  ParallelPVariant=InternalParameters  IdealPVariant=Disabled  IVariant=Disabled  DVariant=Disabled  IntegratorVariant=Disabled  SatVariant=Disabled  AWVariant=Disabled  PCopyVariant=Disabled  TRVariant=Disabled  FdbkBlocksVariant=Forward  IdealPFdbkVariant=Disabled  SatFdbkVariant=Disabled  DerivativeFilterVariant=Disabled  NVariant=Disabled  NCopyVariant=Disabled_SignalSpec  FilterICVariant=Disabled  IntegratorICVariant=Disabled  ExternalResetVariant=Disabled  TRSumVariant=Passthrough  SumFdbkVariant=Disabled  SumVariant=Passthrough_P  TsampFilterVariant=InternalTs  TsampNgainVariant=Passthrough  TsampIntegralVariant=Disabled_SignalSpec  ExternalSaturationOutDataTypeStr=Inherit: Same as second input
  P_CONT_too : pid_lib/PID Controller  Controller=P  Form=Parallel  TimeDomain=Continuous-time  UseExternalTs=off  SampleTime=-1  IntegratorMethod=Forward Euler  FilterMethod=Forward Euler  ControllerParametersSource=internal  P=6  I=0.151389824684851  D=0  UseFilter=on  N=100  TunerSelectOption=Transfer Function Based (PID Tuner App)  InitialConditionSource=internal  InitialConditionForIntegrator=0  InitialConditionForFilter=0  DifferentiatorICPrevScaledInput=0  ExternalReset=none  TrackingMode=off  Kt=1  LimitOutput=off  SatLimitsSource=internal  UpperSaturationLimit=inf  LowerSaturationLimit=-inf  LinearizeAsGain=on  AntiWindupMode=none  Kb=1  POutMin=[]  POutMax=[]  IOutMin=[]  IOutMax=[]  DOutMin=[]  DOutMax=[]  NOutMin=[]  NOutMax=[]  SumOutMin=[]  SumOutMax=[]  SaturationOutMin=[]  SaturationOutMax=[]  PParamMin=[]  PParamMax=[]  IParamMin=[]  IParamMax=[]  DParamMin=[]  DParamMax=[]  NParamMin=[]  NParamMax=[]  KbParamMin=[]  KbParamMax=[]  KtParamMin=[]  KtParamMax=[]  KbOutMin=[]  KbOutMax=[]  KtOutMin=[]  KtOutMax=[]  IntegratorOutMin=[]  IntegratorOutMax=[]  FilterOutMin=[]  FilterOutMax=[]  SumI1OutMin=[]  SumI1OutMax=[]  SumI2OutMin=[]  SumI2OutMax=[]  SumI3OutMin=[]  SumI3OutMax=[]  SumI4OutMin=[]  SumI4OutMax=[]  SumDOutMin=[]  SumDOutMax=[]  DifferentiatorOutMin=[]  DifferentiatorOutMax=[]  FilterDiffOutCoefMin=[]  FilterDiffOutCoefMax=[]  ReciprocalOutMin=[]  ReciprocalOutMax=[]  SumDenOutMin=[]  SumDenOutMax=[]  SumNumOutMin=[]  SumNumOutMax=[]  DivideOutMin=[]  DivideOutMax=[]  UdiffTsProdOutMin=[]  UdiffTsProdOutMax=[]  NTsProdOutMin=[]  NTsProdOutMax=[]  UintegralTsProdOutMin=[]  UintegralTsProdOutMax=[]  UngainTsProdOutMin=[]  UngainTsProdOutMax=[]  IntegratorContinuousStateAttributes=''  IntegratorStateMustResolveToSignalObject=off  IntegratorRTWStateStorageClass=Auto  FilterContinuousStateAttributes=''  FilterStateMustResolveToSignalObject=off  FilterRTWStateStorageClass=Auto  ParallelPVariant=InternalParameters  IdealPVariant=Disabled  IVariant=Disabled  DVariant=Disabled  IntegratorVariant=Disabled  SatVariant=Disabled  AWVariant=Disabled  PCopyVariant=Disabled  TRVariant=Disabled  FdbkBlocksVariant=Forward  IdealPFdbkVariant=Disabled  SatFdbkVariant=Disabled  DerivativeFilterVariant=Disabled  NVariant=Disabled  NCopyVariant=Disabled_SignalSpec  FilterICVariant=Disabled  IntegratorICVariant=Disabled  ExternalResetVariant=Disabled  TRSumVariant=Passthrough  SumFdbkVariant=Disabled  SumVariant=Passthrough_P  TsampFilterVariant=InternalTs  TsampNgainVariant=Passthrough  TsampIntegralVariant=Disabled_SignalSpec  ExternalSaturationOutDataTypeStr=Inherit: Same as second input
  Sum1 : Sum  Inputs=|+-
  Sum3 : Sum  Inputs=|+-
  TQ : Outport
  wires:
  Sum3/1 -> P_CONT/1
  P_CONT/1 -> TQ/1  "TQ"
  ANG_MEAS/1 -> Sum1/2
  ANG_dot_MEAS/1 -> Sum3/2
  Sum1/1 -> P_CONT_too/1
  ANG_CMD/1 -> Sum1/1
  P_CONT_too/1 -> Sum3/1

== system three_a_attitude_control_euler/Attitude control/ROLL control ==
  note: NOTE: 1 radian = 57 degrees
  ANG_CMD : Inport
  ANG_MEAS : Inport  Port=2
  ANG_dot_MEAS : Inport  Port=3
  P_CONT : pid_lib/PID Controller  Controller=P  Form=Parallel  TimeDomain=Continuous-time  UseExternalTs=off  SampleTime=-1  IntegratorMethod=Forward Euler  FilterMethod=Forward Euler  ControllerParametersSource=internal  P=1  I=7.09690484808648  D=-0.334898279224841  UseFilter=on  N=17.076664592689  TunerSelectOption=Transfer Function Based (PID Tuner App)  InitialConditionSource=internal  InitialConditionForIntegrator=0  InitialConditionForFilter=0  DifferentiatorICPrevScaledInput=0  ExternalReset=none  TrackingMode=off  Kt=1  LimitOutput=off  SatLimitsSource=internal  UpperSaturationLimit=inf  LowerSaturationLimit=-inf  LinearizeAsGain=on  AntiWindupMode=none  Kb=1  POutMin=[]  POutMax=[]  IOutMin=[]  IOutMax=[]  DOutMin=[]  DOutMax=[]  NOutMin=[]  NOutMax=[]  SumOutMin=[]  SumOutMax=[]  SaturationOutMin=[]  SaturationOutMax=[]  PParamMin=[]  PParamMax=[]  IParamMin=[]  IParamMax=[]  DParamMin=[]  DParamMax=[]  NParamMin=[]  NParamMax=[]  KbParamMin=[]  KbParamMax=[]  KtParamMin=[]  KtParamMax=[]  KbOutMin=[]  KbOutMax=[]  KtOutMin=[]  KtOutMax=[]  IntegratorOutMin=[]  IntegratorOutMax=[]  FilterOutMin=[]  FilterOutMax=[]  SumI1OutMin=[]  SumI1OutMax=[]  SumI2OutMin=[]  SumI2OutMax=[]  SumI3OutMin=[]  SumI3OutMax=[]  SumI4OutMin=[]  SumI4OutMax=[]  SumDOutMin=[]  SumDOutMax=[]  DifferentiatorOutMin=[]  DifferentiatorOutMax=[]  FilterDiffOutCoefMin=[]  FilterDiffOutCoefMax=[]  ReciprocalOutMin=[]  ReciprocalOutMax=[]  SumDenOutMin=[]  SumDenOutMax=[]  SumNumOutMin=[]  SumNumOutMax=[]  DivideOutMin=[]  DivideOutMax=[]  UdiffTsProdOutMin=[]  UdiffTsProdOutMax=[]  NTsProdOutMin=[]  NTsProdOutMax=[]  UintegralTsProdOutMin=[]  UintegralTsProdOutMax=[]  UngainTsProdOutMin=[]  UngainTsProdOutMax=[]  IntegratorContinuousStateAttributes=''  IntegratorStateMustResolveToSignalObject=off  IntegratorRTWStateStorageClass=Auto  FilterContinuousStateAttributes=''  FilterStateMustResolveToSignalObject=off  FilterRTWStateStorageClass=Auto  ParallelPVariant=InternalParameters  IdealPVariant=Disabled  IVariant=Disabled  DVariant=Disabled  IntegratorVariant=Disabled  SatVariant=Disabled  AWVariant=Disabled  PCopyVariant=Disabled  TRVariant=Disabled  FdbkBlocksVariant=Forward  IdealPFdbkVariant=Disabled  SatFdbkVariant=Disabled  DerivativeFilterVariant=Disabled  NVariant=Disabled  NCopyVariant=Disabled_SignalSpec  FilterICVariant=Disabled  IntegratorICVariant=Disabled  ExternalResetVariant=Disabled  TRSumVariant=Passthrough  SumFdbkVariant=Disabled  SumVariant=Passthrough_P  TsampFilterVariant=InternalTs  TsampNgainVariant=Passthrough  TsampIntegralVariant=Disabled_SignalSpec  ExternalSaturationOutDataTypeStr=Inherit: Same as second input
  P_CONT_too : pid_lib/PID Controller  Controller=P  Form=Parallel  TimeDomain=Continuous-time  UseExternalTs=off  SampleTime=-1  IntegratorMethod=Forward Euler  FilterMethod=Forward Euler  ControllerParametersSource=internal  P=6  I=0.151389824684851  D=0  UseFilter=on  N=100  TunerSelectOption=Transfer Function Based (PID Tuner App)  InitialConditionSource=internal  InitialConditionForIntegrator=0  InitialConditionForFilter=0  DifferentiatorICPrevScaledInput=0  ExternalReset=none  TrackingMode=off  Kt=1  LimitOutput=off  SatLimitsSource=internal  UpperSaturationLimit=inf  LowerSaturationLimit=-inf  LinearizeAsGain=on  AntiWindupMode=none  Kb=1  POutMin=[]  POutMax=[]  IOutMin=[]  IOutMax=[]  DOutMin=[]  DOutMax=[]  NOutMin=[]  NOutMax=[]  SumOutMin=[]  SumOutMax=[]  SaturationOutMin=[]  SaturationOutMax=[]  PParamMin=[]  PParamMax=[]  IParamMin=[]  IParamMax=[]  DParamMin=[]  DParamMax=[]  NParamMin=[]  NParamMax=[]  KbParamMin=[]  KbParamMax=[]  KtParamMin=[]  KtParamMax=[]  KbOutMin=[]  KbOutMax=[]  KtOutMin=[]  KtOutMax=[]  IntegratorOutMin=[]  IntegratorOutMax=[]  FilterOutMin=[]  FilterOutMax=[]  SumI1OutMin=[]  SumI1OutMax=[]  SumI2OutMin=[]  SumI2OutMax=[]  SumI3OutMin=[]  SumI3OutMax=[]  SumI4OutMin=[]  SumI4OutMax=[]  SumDOutMin=[]  SumDOutMax=[]  DifferentiatorOutMin=[]  DifferentiatorOutMax=[]  FilterDiffOutCoefMin=[]  FilterDiffOutCoefMax=[]  ReciprocalOutMin=[]  ReciprocalOutMax=[]  SumDenOutMin=[]  SumDenOutMax=[]  SumNumOutMin=[]  SumNumOutMax=[]  DivideOutMin=[]  DivideOutMax=[]  UdiffTsProdOutMin=[]  UdiffTsProdOutMax=[]  NTsProdOutMin=[]  NTsProdOutMax=[]  UintegralTsProdOutMin=[]  UintegralTsProdOutMax=[]  UngainTsProdOutMin=[]  UngainTsProdOutMax=[]  IntegratorContinuousStateAttributes=''  IntegratorStateMustResolveToSignalObject=off  IntegratorRTWStateStorageClass=Auto  FilterContinuousStateAttributes=''  FilterStateMustResolveToSignalObject=off  FilterRTWStateStorageClass=Auto  ParallelPVariant=InternalParameters  IdealPVariant=Disabled  IVariant=Disabled  DVariant=Disabled  IntegratorVariant=Disabled  SatVariant=Disabled  AWVariant=Disabled  PCopyVariant=Disabled  TRVariant=Disabled  FdbkBlocksVariant=Forward  IdealPFdbkVariant=Disabled  SatFdbkVariant=Disabled  DerivativeFilterVariant=Disabled  NVariant=Disabled  NCopyVariant=Disabled_SignalSpec  FilterICVariant=Disabled  IntegratorICVariant=Disabled  ExternalResetVariant=Disabled  TRSumVariant=Passthrough  SumFdbkVariant=Disabled  SumVariant=Passthrough_P  TsampFilterVariant=InternalTs  TsampNgainVariant=Passthrough  TsampIntegralVariant=Disabled_SignalSpec  ExternalSaturationOutDataTypeStr=Inherit: Same as second input
  Sum1 : Sum  Inputs=|+-
  Sum3 : Sum  Inputs=|+-
  TQ : Outport
  wires:
  Sum3/1 -> P_CONT/1
  P_CONT/1 -> TQ/1  "TQ"
  ANG_MEAS/1 -> Sum1/2
  ANG_dot_MEAS/1 -> Sum3/2
  Sum1/1 -> P_CONT_too/1
  ANG_CMD/1 -> Sum1/1
  P_CONT_too/1 -> Sum3/1

== system three_a_attitude_control_euler/Attitude control/YAW control ==
  Yaw_CMD : Inport
  SUT_BUS : Inport  Port=2
  Bus Selector3 : BusSelector  OutputSignals=phi; theta; psi
  Bus Selector4 : BusSelector  OutputSignals=dphi; dtheta; dpsi
  FINAL_DES_YAW_CONTROL_SYSTEM : Subsystem
  Selector2 : Selector  InputPortWidth=3  IndexOptions=Index vector (dialog)  Indices=3  OutputSizes=1
  Selector3 : Selector  InputPortWidth=3  IndexOptions=Index vector (dialog)  Indices=3  OutputSizes=1
  TQ_Yaw : Outport  VectorParamsAs1DForOutWhenUnconnected=off
  wires:
  Selector2/1 -> FINAL_DES_YAW_CONTROL_SYSTEM/2(YAW_MEAS)
  Yaw_CMD/1 -> FINAL_DES_YAW_CONTROL_SYSTEM/1(YAW_CMD)
  Selector3/1 -> FINAL_DES_YAW_CONTROL_SYSTEM/3(YAW_dot_MEAS)
  FINAL_DES_YAW_CONTROL_SYSTEM/1(TQ_YAW) -> TQ_Yaw/1  "TQ_Z_YAW"
  Bus Selector4/1 -> Selector3/1  "<dphi; dtheta; dpsi>"
  Bus Selector3/1 -> Selector2/1  "<phi; theta; psi>"
  SUT_BUS/1 -> Bus Selector4/1, Bus Selector3/1

== system three_a_attitude_control_euler/Attitude control/psi ==
  In1 : Inport
  Bus Selector1 : BusSelector  OutputSignals=phi; theta; psi
  Bus Selector2 : BusSelector  OutputSignals=dphi; dtheta; dpsi
  Selector1 : Selector  InputPortWidth=3  IndexOptions=Index vector (dialog)  Indices=1  OutputSizes=1
  Selector2 : Selector  InputPortWidth=3  IndexOptions=Index vector (dialog)  Indices=1  OutputSizes=1
  ANG_MEAS : Outport  VectorParamsAs1DForOutWhenUnconnected=off
  Out2 : Outport  Port=2  VectorParamsAs1DForOutWhenUnconnected=off
  wires:
  In1/1 -> Bus Selector2/1, Bus Selector1/1
  Selector1/1 -> ANG_MEAS/1
  Bus Selector1/1 -> Selector1/1  "<phi; theta; psi>"
  Bus Selector2/1 -> Selector2/1  "<dphi; dtheta; dpsi>"
  Selector2/1 -> Out2/1

== system three_a_attitude_control_euler/Attitude control/theta ==
  In1 : Inport
  Bus Selector1 : BusSelector  OutputSignals=phi; theta; psi
  Bus Selector2 : BusSelector  OutputSignals=dphi; dtheta; dpsi
  Selector1 : Selector  InputPortWidth=3  IndexOptions=Index vector (dialog)  Indices=2  OutputSizes=1
  Selector2 : Selector  InputPortWidth=3  IndexOptions=Index vector (dialog)  Indices=2  OutputSizes=1
  ANG_MEAS : Outport  VectorParamsAs1DForOutWhenUnconnected=off
  ANG_dot_MEAS : Outport  Port=2  VectorParamsAs1DForOutWhenUnconnected=off
  wires:
  In1/1 -> Bus Selector2/1, Bus Selector1/1
  Selector1/1 -> ANG_MEAS/1
  Bus Selector1/1 -> Selector1/1  "<phi; theta; psi>"
  Bus Selector2/1 -> Selector2/1  "<dphi; dtheta; dpsi>"
  Selector2/1 -> ANG_dot_MEAS/1

== system three_a_attitude_control_euler/Commands/Acro ==
  Demux : Demux  Tag=STV Demux
      settings: DisplayOption=none
  FromWs : FromWorkspace  Tag=STV FromWs  VariableName=tuvar
      SigBuilderData=|
      | common.afterFinalStr = 'Extrapolate'
      | common.sampleTime = 0
      | dataSet(1).timeRange = [0 200]
      | dataSet(1).name = 'small_steps'
      | dataSet(2).timeRange = [0 200]
      | dataSet(2).name = 'zStairs_xyConstVEL'
      | dataSet(3).timeRange = [0 500]
      | dataSet(3).name = 'sineWaves'
      | dataSet(4).timeRange = [0 200]
      | dataSet(4).name = 'ZERO'
      | dataSet(5).timeRange = [0 200]
      | dataSet(5).name = 'SEARCH_P1'
      | sbobj.Name = 'Signal Builder'
      | sbobj.Groups(1).Name = 'small_steps'
      | sbobj.Groups(1).Signals(1).Name = 'Z'
      | sbobj.Groups(1).Signals(1).XData = [0 10 10.000001 20 20.000001 30 30.000001 55 200]
      | sbobj.Groups(1).Signals(1).YData = [0 0 2 2 2 2 2 2 2]
      | sbobj.Groups(1).Signals(2).Name = 'roll'
      | sbobj.Groups(1).Signals(2).XData = [0 10 10.000001 20 20.000001 30 30.000001 55 200]
      | sbobj.Groups(1).Signals(2).YData = [0 0 0 0 3 3 3 3 3]
      | sbobj.Groups(1).Signals(3).Name = 'pitch'
      | sbobj.Groups(1).Signals(3).XData = [0 10 10.000001 20 20.000001 30 30.000001 55 200]
      | sbobj.Groups(1).Signals(3).YData = [0 0 0 0 0 0 1 1 1]
      | sbobj.Groups(1).Signals(4).Name = 'Yaw'
      | sbobj.Groups(1).Signals(4).XData = [0 200]
      | sbobj.Groups(1).Signals(4).YData = [0 0]
      | sbobj.Groups(1).TimeRange = [0 200]
      | sbobj.Groups(2).Name = 'zStairs_xyConstVEL'
      | sbobj.Groups(2).Signals(1).Name = 'Z'
      | sbobj.Groups(2).Signals(1).XData = [0 10 10.000001 20 20.000001 30 30.000001 40 40.000001 55 200]
      | sbobj.Groups(2).Signals(1).YData = [0 0 1 1 2 2 1 1 0 0 0]
      | sbobj.Groups(2).Signals(2).Name = 'roll'
      | sbobj.Groups(2).Signals(2).XData = [0 10 10.000001 20 20.000001 30 30.000001 40 40.000001 55 200]
      | sbobj.Groups(2).Signals(2).YData = [0 1 1.0000001 2 2.0000001 3 3.0000001 4 4.0000001 5.5 20]
      | sbobj.Groups(2).Signals(3).Name = 'pitch'
      | sbobj.Groups(2).Signals(3).XData = [0 10 10.000001 20 20.000001 30 30.000001 40 40.000001 55 200]
      | sbobj.Groups(2).Signals(3).YData = [0 0.5 0.50000005 1 1.00000005 1.5 1.50000005 2 2.00000005 2.75 10]
      | sbobj.Groups(2).Signals(4).Name = 'Yaw'
      | sbobj.Groups(2).Signals(4).XData = [0 200]
      | sbobj.Groups(2).Signals(4).YData = [0 0]
      | sbobj.Groups(2).TimeRange = [0 200]
      | sbobj.Groups(3).Name = 'sineWaves'
      | sbobj.Groups(3).Signals(1).Name = 'Z'
      | sbobj.Groups(3).Signals(1).XData = [0 0.1 0.2 0.3 0.4 0.5 0.6 0.7 0.8 0.9 1 1.1 ... (5001 elements, 1x5001)]
      | sbobj.Groups(3).Signals(1).YData = [0 0.0314107325553 0.0627904665622 0.0941082340641 0.125333128258 0.156434333994 0.18738115819 0.218143060119 0.248689681547 0.278990876699 0.309016742004 0.338737645607 ... (5001 elements, 1x5001)]
      | sbobj.Groups(3).Signals(2).Name = 'roll'
      | sbobj.Groups(3).Signals(2).XData = [0 0.1 0.2 0.3 0.4 0.5 0.6 0.7 0.8 0.9 1 1.1 ... (5001 elements, 1x5001)]
      | sbobj.Groups(3).Signals(2).YData = [0 0.01 0.02 0.03 0.04 0.05 0.06 0.07 0.08 0.09 0.1 0.11 ... (5001 elements, 1x5001)]
      | sbobj.Groups(3).Signals(3).Name = 'pitch'
      | sbobj.Groups(3).Signals(3).XData = [0 0.1 0.2 0.3 0.4 0.5 0.6 0.7 0.8 0.9 1 1.1 ... (5001 elements, 1x5001)]
      | sbobj.Groups(3).Signals(3).YData = [0 0.0157073040455 0.0314107325553 0.04710641095 0.0627904665622 0.0784590295926 0.0941082340641 0.109734218776 0.125333128258 0.140901113717 0.156434333994 0.171928956505 ... (5001 elements, 1x5001)]
      | sbobj.Groups(3).Signals(4).Name = 'Yaw'
      | sbobj.Groups(3).Signals(4).XData = [0 500]
      | sbobj.Groups(3).Signals(4).YData = [0 0]
      | sbobj.Groups(3).TimeRange = [0 500]
      | sbobj.Groups(4).Name = 'ZERO'
      | sbobj.Groups(4).Signals(1).Name = 'Z'
      | sbobj.Groups(4).Signals(1).XData = [0 200]
      | sbobj.Groups(4).Signals(1).YData = [0 0]
      | sbobj.Groups(4).Signals(2).Name = 'roll'
      | sbobj.Groups(4).Signals(2).XData = [0 200]
      | sbobj.Groups(4).Signals(2).YData = [0 0]
      | sbobj.Groups(4).Signals(3).Name = 'pitch'
      | sbobj.Groups(4).Signals(3).XData = [0 200]
      | sbobj.Groups(4).Signals(3).YData = [0 0]
      | sbobj.Groups(4).Signals(4).Name = 'Yaw'
      | sbobj.Groups(4).Signals(4).XData = [0 200]
      | sbobj.Groups(4).Signals(4).YData = [0 0]
      | sbobj.Groups(4).TimeRange = [0 200]
      | sbobj.Groups(5).Name = 'SEARCH_P1'
      | sbobj.Groups(5).Signals(1).Name = 'Z'
      | sbobj.Groups(5).Signals(1).XData = [0 7 27 32 52 57 77 82 102 107 127 132 157 187 200]
      | sbobj.Groups(5).Signals(1).YData = [0 5 5 5 5 5 5 5 5 5 5 5 5 0 0]
      | sbobj.Groups(5).Signals(2).Name = 'roll'
      | sbobj.Groups(5).Signals(2).XData = [0 200]
      | sbobj.Groups(5).Signals(2).YData = [0 0]
      | sbobj.Groups(5).Signals(3).Name = 'pitch'
      | sbobj.Groups(5).Signals(3).XData = [0 3.44827586207 6.89655172414 10.3448275862 13.7931034483 17.2413793103 20.6896551724 24.1379310345 27.5862068966 31.0344827586 34.4827586207 37.9310344828 41.3793103448 44.8275862069 48.275862069 51.724137931 55.1724137931 58.6206896552 62.0689655172 65.5172413793 68.9655172414 72.4137931034 75.8620689655 79.3103448276 82.7586206897 86.2068965517 89.6551724138 93.1034482759 96.5517241379 100 103.448275862 106.896551724 110.344827586 113.793103448 117.24137931 120.689655172 124.137931034 127.586206897 131.034482759 134.482758621 137.931034483 141.379310345 144.827586207 148.275862069 151.724137931 155.172413793 158.620689655 162.068965517 165.517241379 168.965517241 172.413793103 175.862068966 179.310344828 182.75862069 186.206896552 189.655172414 193.103448276 196.551724138 200]
      | sbobj.Groups(5).Signals(3).YData = [0 38.694679238 75.5800382808 108.931358735 137.189169923 159.032168 173.438998653 179.736014493 177.628774057 167.215809567 148.984019668 123.785902594 92.7996942919 57.4742754245 19.4614233163 -19.4614233163 -57.4742754245 -92.7996942919 -123.785902594 -148.984019668 -167.215809567 -177.628774057 -179.736014493 -173.438998653 -159.032168 -137.189169923 -108.931358735 -75.5800382808 -38.694679238 0 38.694679238 75.5800382808 108.931358735 137.189169923 159.032168 173.438998653 179.736014493 177.628774057 167.215809567 148.984019668 123.785902594 92.7996942919 57.4742754245 19.4614233163 -19.4614233163 -57.4742754245 -92.7996942919 -123.785902594 -148.984019668 -167.215809567 -177.628774057 -179.736014493 -173.438998653 -159.032168 -137.189169923 -108.931358735 -75.5800382808 -38.694679238 0]
      | sbobj.Groups(5).Signals(4).Name = 'Yaw'
      | sbobj.Groups(5).Signals(4).XData = [0 200]
      | sbobj.Groups(5).Signals(4).YData = [0 0]
      | sbobj.Groups(5).TimeRange = [0 200]
  Z : Outport  VectorParamsAs1DForOutWhenUnconnected=off
  roll : Outport  Tag=STV Outport  Port=2  VectorParamsAs1DForOutWhenUnconnected=off
  pitch : Outport  Tag=STV Outport  Port=3  VectorParamsAs1DForOutWhenUnconnected=off
  Yaw : Outport  Tag=STV Outport  Port=4
  wires:
  Demux/1 -> Z/1
  FromWs/1 -> Demux/1
  Demux/2 -> roll/1
  Demux/3 -> pitch/1
  Demux/4 -> Yaw/1

== system three_a_attitude_control_euler/Commands/Altitude  ==
  Demux : Demux  Tag=STV Demux
      settings: DisplayOption=none
  FromWs : FromWorkspace  Tag=STV FromWs  VariableName=tuvar
      SigBuilderData=|
      | common.afterFinalStr = 'Extrapolate'
      | common.sampleTime = 0
      | dataSet(1).timeRange = [0 200]
      | dataSet(1).name = 'small_steps'
      | dataSet(2).timeRange = [0 200]
      | dataSet(2).name = 'zStairs_xyConstVEL'
      | dataSet(3).timeRange = [0 500]
      | dataSet(3).name = 'sineWaves'
      | dataSet(4).timeRange = [0 200]
      | dataSet(4).name = 'ZERO'
      | dataSet(5).timeRange = [0 200]
      | dataSet(5).name = 'SEARCH_P1'
      | sbobj.Name = 'Signal Builder'
      | sbobj.Groups(1).Name = 'small_steps'
      | sbobj.Groups(1).Signals(1).Name = 'Z'
      | sbobj.Groups(1).Signals(1).XData = [0 10 10.000001 20 20.000001 30 30.000001 55 200]
      | sbobj.Groups(1).Signals(1).YData = [0 0 2 2 2 2 2 2 2]
      | sbobj.Groups(1).Signals(2).Name = 'roll'
      | sbobj.Groups(1).Signals(2).XData = [0 10 10.000001 20 20.000001 30 30.000001 55 200]
      | sbobj.Groups(1).Signals(2).YData = [0 0 0 0 3 3 3 3 3]
      | sbobj.Groups(1).Signals(3).Name = 'pitch'
      | sbobj.Groups(1).Signals(3).XData = [0 10 10.000001 20 20.000001 30 30.000001 55 200]
      | sbobj.Groups(1).Signals(3).YData = [0 0 0 0 0 0 1 1 1]
      | sbobj.Groups(1).Signals(4).Name = 'Yaw'
      | sbobj.Groups(1).Signals(4).XData = [0 200]
      | sbobj.Groups(1).Signals(4).YData = [0 0]
      | sbobj.Groups(1).TimeRange = [0 200]
      | sbobj.Groups(2).Name = 'zStairs_xyConstVEL'
      | sbobj.Groups(2).Signals(1).Name = 'Z'
      | sbobj.Groups(2).Signals(1).XData = [0 10 10.000001 20 20.000001 30 30.000001 40 40.000001 55 200]
      | sbobj.Groups(2).Signals(1).YData = [0 0 1 1 2 2 1 1 0 0 0]
      | sbobj.Groups(2).Signals(2).Name = 'roll'
      | sbobj.Groups(2).Signals(2).XData = [0 10 10.000001 20 20.000001 30 30.000001 40 40.000001 55 200]
      | sbobj.Groups(2).Signals(2).YData = [0 1 1.0000001 2 2.0000001 3 3.0000001 4 4.0000001 5.5 20]
      | sbobj.Groups(2).Signals(3).Name = 'pitch'
      | sbobj.Groups(2).Signals(3).XData = [0 10 10.000001 20 20.000001 30 30.000001 40 40.000001 55 200]
      | sbobj.Groups(2).Signals(3).YData = [0 0.5 0.50000005 1 1.00000005 1.5 1.50000005 2 2.00000005 2.75 10]
      | sbobj.Groups(2).Signals(4).Name = 'Yaw'
      | sbobj.Groups(2).Signals(4).XData = [0 200]
      | sbobj.Groups(2).Signals(4).YData = [0 0]
      | sbobj.Groups(2).TimeRange = [0 200]
      | sbobj.Groups(3).Name = 'sineWaves'
      | sbobj.Groups(3).Signals(1).Name = 'Z'
      | sbobj.Groups(3).Signals(1).XData = [0 0.1 0.2 0.3 0.4 0.5 0.6 0.7 0.8 0.9 1 1.1 ... (5001 elements, 1x5001)]
      | sbobj.Groups(3).Signals(1).YData = [0 0.0314107325553 0.0627904665622 0.0941082340641 0.125333128258 0.156434333994 0.18738115819 0.218143060119 0.248689681547 0.278990876699 0.309016742004 0.338737645607 ... (5001 elements, 1x5001)]
      | sbobj.Groups(3).Signals(2).Name = 'roll'
      | sbobj.Groups(3).Signals(2).XData = [0 0.1 0.2 0.3 0.4 0.5 0.6 0.7 0.8 0.9 1 1.1 ... (5001 elements, 1x5001)]
      | sbobj.Groups(3).Signals(2).YData = [0 0.01 0.02 0.03 0.04 0.05 0.06 0.07 0.08 0.09 0.1 0.11 ... (5001 elements, 1x5001)]
      | sbobj.Groups(3).Signals(3).Name = 'pitch'
      | sbobj.Groups(3).Signals(3).XData = [0 0.1 0.2 0.3 0.4 0.5 0.6 0.7 0.8 0.9 1 1.1 ... (5001 elements, 1x5001)]
      | sbobj.Groups(3).Signals(3).YData = [0 0.0157073040455 0.0314107325553 0.04710641095 0.0627904665622 0.0784590295926 0.0941082340641 0.109734218776 0.125333128258 0.140901113717 0.156434333994 0.171928956505 ... (5001 elements, 1x5001)]
      | sbobj.Groups(3).Signals(4).Name = 'Yaw'
      | sbobj.Groups(3).Signals(4).XData = [0 500]
      | sbobj.Groups(3).Signals(4).YData = [0 0]
      | sbobj.Groups(3).TimeRange = [0 500]
      | sbobj.Groups(4).Name = 'ZERO'
      | sbobj.Groups(4).Signals(1).Name = 'Z'
      | sbobj.Groups(4).Signals(1).XData = [0 200]
      | sbobj.Groups(4).Signals(1).YData = [0 0]
      | sbobj.Groups(4).Signals(2).Name = 'roll'
      | sbobj.Groups(4).Signals(2).XData = [0 200]
      | sbobj.Groups(4).Signals(2).YData = [0 0]
      | sbobj.Groups(4).Signals(3).Name = 'pitch'
      | sbobj.Groups(4).Signals(3).XData = [0 200]
      | sbobj.Groups(4).Signals(3).YData = [0 0]
      | sbobj.Groups(4).Signals(4).Name = 'Yaw'
      | sbobj.Groups(4).Signals(4).XData = [0 200]
      | sbobj.Groups(4).Signals(4).YData = [0 0]
      | sbobj.Groups(4).TimeRange = [0 200]
      | sbobj.Groups(5).Name = 'SEARCH_P1'
      | sbobj.Groups(5).Signals(1).Name = 'Z'
      | sbobj.Groups(5).Signals(1).XData = [0 5 5 10 10 15 15 20 20 25 30 30 35 40 40 45 45 50 50 55 55 60 60 65 65 70 70 75 75 80 80 85 85 90 90 95 95 100 100 105 105 110 110 115 115 120 120 125 125 130 130 135 135 140 140 145 145 150 150 155 155 160 160 165 165 170 170 175 175 180 180 185 185 190 190 195 195 200]
      | sbobj.Groups(5).Signals(1).YData = [0 0 0.9 0.9 2 2 4.1 4.1 0 0 0 4 4 4 2 2 0 0 2 2 0 0 2 2 0 0 2 2 0 0 2 2 0 0 2 2 0 0 2 2 0 0 2 2 0 0 2 2 0 0 2 2 0 0 2 2 0 0 2 2 0 0 2 2 0 0 2 2 0 0 2 2 0 0 2 2 0 0]
      | sbobj.Groups(5).Signals(2).Name = 'roll'
      | sbobj.Groups(5).Signals(2).XData = [0 200]
      | sbobj.Groups(5).Signals(2).YData = [0 0]
      | sbobj.Groups(5).Signals(3).Name = 'pitch'
      | sbobj.Groups(5).Signals(3).XData = [0 200]
      | sbobj.Groups(5).Signals(3).YData = [0 0]
      | sbobj.Groups(5).Signals(4).Name = 'Yaw'
      | sbobj.Groups(5).Signals(4).XData = [0 200]
      | sbobj.Groups(5).Signals(4).YData = [0 0]
      | sbobj.Groups(5).TimeRange = [0 200]
  Z : Outport  VectorParamsAs1DForOutWhenUnconnected=off
  roll : Outport  Tag=STV Outport  Port=2  VectorParamsAs1DForOutWhenUnconnected=off
  pitch : Outport  Tag=STV Outport  Port=3  VectorParamsAs1DForOutWhenUnconnected=off
  Yaw : Outport  Tag=STV Outport  Port=4
  wires:
  Demux/1 -> Z/1
  FromWs/1 -> Demux/1
  Demux/2 -> roll/1
  Demux/3 -> pitch/1
  Demux/4 -> Yaw/1

== system three_a_attitude_control_euler/Commands/Ground ==
  Demux : Demux  Tag=STV Demux
      settings: DisplayOption=none
  FromWs : FromWorkspace  Tag=STV FromWs  VariableName=tuvar
      SigBuilderData=|
      | common.afterFinalStr = 'Extrapolate'
      | common.sampleTime = 0
      | dataSet(1).timeRange = [0 200]
      | dataSet(1).name = 'small_steps'
      | dataSet(2).timeRange = [0 200]
      | dataSet(2).name = 'zStairs_xyConstVEL'
      | dataSet(3).timeRange = [0 500]
      | dataSet(3).name = 'sineWaves'
      | dataSet(4).timeRange = [0 200]
      | dataSet(4).name = 'ZERO'
      | dataSet(5).timeRange = [0 200]
      | dataSet(5).name = 'SEARCH_P1'
      | sbobj.Name = 'Signal Builder'
      | sbobj.Groups(1).Name = 'small_steps'
      | sbobj.Groups(1).Signals(1).Name = 'Z'
      | sbobj.Groups(1).Signals(1).XData = [0 10 10.000001 20 20.000001 30 30.000001 55 200]
      | sbobj.Groups(1).Signals(1).YData = [0 0 2 2 2 2 2 2 2]
      | sbobj.Groups(1).Signals(2).Name = 'roll'
      | sbobj.Groups(1).Signals(2).XData = [0 10 10.000001 20 20.000001 30 30.000001 55 200]
      | sbobj.Groups(1).Signals(2).YData = [0 0 0 0 3 3 3 3 3]
      | sbobj.Groups(1).Signals(3).Name = 'pitch'
      | sbobj.Groups(1).Signals(3).XData = [0 10 10.000001 20 20.000001 30 30.000001 55 200]
      | sbobj.Groups(1).Signals(3).YData = [0 0 0 0 0 0 1 1 1]
      | sbobj.Groups(1).Signals(4).Name = 'Yaw'
      | sbobj.Groups(1).Signals(4).XData = [0 200]
      | sbobj.Groups(1).Signals(4).YData = [0 0]
      | sbobj.Groups(1).TimeRange = [0 200]
      | sbobj.Groups(2).Name = 'zStairs_xyConstVEL'
      | sbobj.Groups(2).Signals(1).Name = 'Z'
      | sbobj.Groups(2).Signals(1).XData = [0 10 10.000001 20 20.000001 30 30.000001 40 40.000001 55 200]
      | sbobj.Groups(2).Signals(1).YData = [0 0 1 1 2 2 1 1 0 0 0]
      | sbobj.Groups(2).Signals(2).Name = 'roll'
      | sbobj.Groups(2).Signals(2).XData = [0 10 10.000001 20 20.000001 30 30.000001 40 40.000001 55 200]
      | sbobj.Groups(2).Signals(2).YData = [0 1 1.0000001 2 2.0000001 3 3.0000001 4 4.0000001 5.5 20]
      | sbobj.Groups(2).Signals(3).Name = 'pitch'
      | sbobj.Groups(2).Signals(3).XData = [0 10 10.000001 20 20.000001 30 30.000001 40 40.000001 55 200]
      | sbobj.Groups(2).Signals(3).YData = [0 0.5 0.50000005 1 1.00000005 1.5 1.50000005 2 2.00000005 2.75 10]
      | sbobj.Groups(2).Signals(4).Name = 'Yaw'
      | sbobj.Groups(2).Signals(4).XData = [0 200]
      | sbobj.Groups(2).Signals(4).YData = [0 0]
      | sbobj.Groups(2).TimeRange = [0 200]
      | sbobj.Groups(3).Name = 'sineWaves'
      | sbobj.Groups(3).Signals(1).Name = 'Z'
      | sbobj.Groups(3).Signals(1).XData = [0 0.1 0.2 0.3 0.4 0.5 0.6 0.7 0.8 0.9 1 1.1 ... (5001 elements, 1x5001)]
      | sbobj.Groups(3).Signals(1).YData = [0 0.0314107325553 0.0627904665622 0.0941082340641 0.125333128258 0.156434333994 0.18738115819 0.218143060119 0.248689681547 0.278990876699 0.309016742004 0.338737645607 ... (5001 elements, 1x5001)]
      | sbobj.Groups(3).Signals(2).Name = 'roll'
      | sbobj.Groups(3).Signals(2).XData = [0 0.1 0.2 0.3 0.4 0.5 0.6 0.7 0.8 0.9 1 1.1 ... (5001 elements, 1x5001)]
      | sbobj.Groups(3).Signals(2).YData = [0 0.01 0.02 0.03 0.04 0.05 0.06 0.07 0.08 0.09 0.1 0.11 ... (5001 elements, 1x5001)]
      | sbobj.Groups(3).Signals(3).Name = 'pitch'
      | sbobj.Groups(3).Signals(3).XData = [0 0.1 0.2 0.3 0.4 0.5 0.6 0.7 0.8 0.9 1 1.1 ... (5001 elements, 1x5001)]
      | sbobj.Groups(3).Signals(3).YData = [0 0.0157073040455 0.0314107325553 0.04710641095 0.0627904665622 0.0784590295926 0.0941082340641 0.109734218776 0.125333128258 0.140901113717 0.156434333994 0.171928956505 ... (5001 elements, 1x5001)]
      | sbobj.Groups(3).Signals(4).Name = 'Yaw'
      | sbobj.Groups(3).Signals(4).XData = [0 500]
      | sbobj.Groups(3).Signals(4).YData = [0 0]
      | sbobj.Groups(3).TimeRange = [0 500]
      | sbobj.Groups(4).Name = 'ZERO'
      | sbobj.Groups(4).Signals(1).Name = 'Z'
      | sbobj.Groups(4).Signals(1).XData = [0 200]
      | sbobj.Groups(4).Signals(1).YData = [0 0]
      | sbobj.Groups(4).Signals(2).Name = 'roll'
      | sbobj.Groups(4).Signals(2).XData = [0 200]
      | sbobj.Groups(4).Signals(2).YData = [0 0]
      | sbobj.Groups(4).Signals(3).Name = 'pitch'
      | sbobj.Groups(4).Signals(3).XData = [0 200]
      | sbobj.Groups(4).Signals(3).YData = [0 0]
      | sbobj.Groups(4).Signals(4).Name = 'Yaw'
      | sbobj.Groups(4).Signals(4).XData = [0 200]
      | sbobj.Groups(4).Signals(4).YData = [0 0]
      | sbobj.Groups(4).TimeRange = [0 200]
      | sbobj.Groups(5).Name = 'SEARCH_P1'
      | sbobj.Groups(5).Signals(1).Name = 'Z'
      | sbobj.Groups(5).Signals(1).XData = [0 200]
      | sbobj.Groups(5).Signals(1).YData = [0 0]
      | sbobj.Groups(5).Signals(2).Name = 'roll'
      | sbobj.Groups(5).Signals(2).XData = [0 200]
      | sbobj.Groups(5).Signals(2).YData = [0 0]
      | sbobj.Groups(5).Signals(3).Name = 'pitch'
      | sbobj.Groups(5).Signals(3).XData = [0 200]
      | sbobj.Groups(5).Signals(3).YData = [0 0]
      | sbobj.Groups(5).Signals(4).Name = 'Yaw'
      | sbobj.Groups(5).Signals(4).XData = [0 200]
      | sbobj.Groups(5).Signals(4).YData = [0 0]
      | sbobj.Groups(5).TimeRange = [0 200]
  Z : Outport  VectorParamsAs1DForOutWhenUnconnected=off
  roll : Outport  Tag=STV Outport  Port=2  VectorParamsAs1DForOutWhenUnconnected=off
  pitch : Outport  Tag=STV Outport  Port=3  VectorParamsAs1DForOutWhenUnconnected=off
  Yaw : Outport  Tag=STV Outport  Port=4
  wires:
  Demux/1 -> Z/1
  FromWs/1 -> Demux/1
  Demux/2 -> roll/1
  Demux/3 -> pitch/1
  Demux/4 -> Yaw/1

== system three_a_attitude_control_euler/Commands/Pitch ==
  Demux : Demux  Tag=STV Demux
      settings: DisplayOption=none
  FromWs : FromWorkspace  Tag=STV FromWs  VariableName=tuvar
      SigBuilderData=|
      | common.afterFinalStr = 'Extrapolate'
      | common.sampleTime = 0
      | dataSet(1).timeRange = [0 200]
      | dataSet(1).name = 'small_steps'
      | dataSet(2).timeRange = [0 200]
      | dataSet(2).name = 'zStairs_xyConstVEL'
      | dataSet(3).timeRange = [0 500]
      | dataSet(3).name = 'sineWaves'
      | dataSet(4).timeRange = [0 200]
      | dataSet(4).name = 'ZERO'
      | dataSet(5).timeRange = [0 200]
      | dataSet(5).name = 'SEARCH_P1'
      | sbobj.Name = 'Signal Builder'
      | sbobj.Groups(1).Name = 'small_steps'
      | sbobj.Groups(1).Signals(1).Name = 'Z'
      | sbobj.Groups(1).Signals(1).XData = [0 10 10.000001 20 20.000001 30 30.000001 55 200]
      | sbobj.Groups(1).Signals(1).YData = [0 0 2 2 2 2 2 2 2]
      | sbobj.Groups(1).Signals(2).Name = 'roll'
      | sbobj.Groups(1).Signals(2).XData = [0 10 10.000001 20 20.000001 30 30.000001 55 200]
      | sbobj.Groups(1).Signals(2).YData = [0 0 0 0 3 3 3 3 3]
      | sbobj.Groups(1).Signals(3).Name = 'pitch'
      | sbobj.Groups(1).Signals(3).XData = [0 10 10.000001 20 20.000001 30 30.000001 55 200]
      | sbobj.Groups(1).Signals(3).YData = [0 0 0 0 0 0 1 1 1]
      | sbobj.Groups(1).Signals(4).Name = 'Yaw'
      | sbobj.Groups(1).Signals(4).XData = [0 200]
      | sbobj.Groups(1).Signals(4).YData = [0 0]
      | sbobj.Groups(1).TimeRange = [0 200]
      | sbobj.Groups(2).Name = 'zStairs_xyConstVEL'
      | sbobj.Groups(2).Signals(1).Name = 'Z'
      | sbobj.Groups(2).Signals(1).XData = [0 10 10.000001 20 20.000001 30 30.000001 40 40.000001 55 200]
      | sbobj.Groups(2).Signals(1).YData = [0 0 1 1 2 2 1 1 0 0 0]
      | sbobj.Groups(2).Signals(2).Name = 'roll'
      | sbobj.Groups(2).Signals(2).XData = [0 10 10.000001 20 20.000001 30 30.000001 40 40.000001 55 200]
      | sbobj.Groups(2).Signals(2).YData = [0 1 1.0000001 2 2.0000001 3 3.0000001 4 4.0000001 5.5 20]
      | sbobj.Groups(2).Signals(3).Name = 'pitch'
      | sbobj.Groups(2).Signals(3).XData = [0 10 10.000001 20 20.000001 30 30.000001 40 40.000001 55 200]
      | sbobj.Groups(2).Signals(3).YData = [0 0.5 0.50000005 1 1.00000005 1.5 1.50000005 2 2.00000005 2.75 10]
      | sbobj.Groups(2).Signals(4).Name = 'Yaw'
      | sbobj.Groups(2).Signals(4).XData = [0 200]
      | sbobj.Groups(2).Signals(4).YData = [0 0]
      | sbobj.Groups(2).TimeRange = [0 200]
      | sbobj.Groups(3).Name = 'sineWaves'
      | sbobj.Groups(3).Signals(1).Name = 'Z'
      | sbobj.Groups(3).Signals(1).XData = [0 0.1 0.2 0.3 0.4 0.5 0.6 0.7 0.8 0.9 1 1.1 ... (5001 elements, 1x5001)]
      | sbobj.Groups(3).Signals(1).YData = [0 0.0314107325553 0.0627904665622 0.0941082340641 0.125333128258 0.156434333994 0.18738115819 0.218143060119 0.248689681547 0.278990876699 0.309016742004 0.338737645607 ... (5001 elements, 1x5001)]
      | sbobj.Groups(3).Signals(2).Name = 'roll'
      | sbobj.Groups(3).Signals(2).XData = [0 0.1 0.2 0.3 0.4 0.5 0.6 0.7 0.8 0.9 1 1.1 ... (5001 elements, 1x5001)]
      | sbobj.Groups(3).Signals(2).YData = [0 0.01 0.02 0.03 0.04 0.05 0.06 0.07 0.08 0.09 0.1 0.11 ... (5001 elements, 1x5001)]
      | sbobj.Groups(3).Signals(3).Name = 'pitch'
      | sbobj.Groups(3).Signals(3).XData = [0 0.1 0.2 0.3 0.4 0.5 0.6 0.7 0.8 0.9 1 1.1 ... (5001 elements, 1x5001)]
      | sbobj.Groups(3).Signals(3).YData = [0 0.0157073040455 0.0314107325553 0.04710641095 0.0627904665622 0.0784590295926 0.0941082340641 0.109734218776 0.125333128258 0.140901113717 0.156434333994 0.171928956505 ... (5001 elements, 1x5001)]
      | sbobj.Groups(3).Signals(4).Name = 'Yaw'
      | sbobj.Groups(3).Signals(4).XData = [0 500]
      | sbobj.Groups(3).Signals(4).YData = [0 0]
      | sbobj.Groups(3).TimeRange = [0 500]
      | sbobj.Groups(4).Name = 'ZERO'
      | sbobj.Groups(4).Signals(1).Name = 'Z'
      | sbobj.Groups(4).Signals(1).XData = [0 200]
      | sbobj.Groups(4).Signals(1).YData = [0 0]
      | sbobj.Groups(4).Signals(2).Name = 'roll'
      | sbobj.Groups(4).Signals(2).XData = [0 200]
      | sbobj.Groups(4).Signals(2).YData = [0 0]
      | sbobj.Groups(4).Signals(3).Name = 'pitch'
      | sbobj.Groups(4).Signals(3).XData = [0 200]
      | sbobj.Groups(4).Signals(3).YData = [0 0]
      | sbobj.Groups(4).Signals(4).Name = 'Yaw'
      | sbobj.Groups(4).Signals(4).XData = [0 200]
      | sbobj.Groups(4).Signals(4).YData = [0 0]
      | sbobj.Groups(4).TimeRange = [0 200]
      | sbobj.Groups(5).Name = 'SEARCH_P1'
      | sbobj.Groups(5).Signals(1).Name = 'Z'
      | sbobj.Groups(5).Signals(1).XData = [0 9.9 200]
      | sbobj.Groups(5).Signals(1).YData = [0 0 0]
      | sbobj.Groups(5).Signals(2).Name = 'roll'
      | sbobj.Groups(5).Signals(2).XData = [0 200]
      | sbobj.Groups(5).Signals(2).YData = [0 0]
      | sbobj.Groups(5).Signals(3).Name = 'pitch'
      | sbobj.Groups(5).Signals(3).XData = [0 0.689655172414 1.37931034483 2.06896551724 2.75862068966 3.44827586207 4.13793103448 4.8275862069 5.51724137931 6.20689655172 6.89655172414 7.58620689655 ... (291 elements, 1x291)]
      | sbobj.Groups(5).Signals(3).YData = [0 5.37426100528 10.497227539 15.1293553798 19.0540513782 22.0878011112 24.088749813 24.9633353463 24.6706630635 23.2244179954 20.6922249539 17.1924864713 ... (291 elements, 1x291)]
      | sbobj.Groups(5).Signals(4).Name = 'Yaw'
      | sbobj.Groups(5).Signals(4).XData = [0 200]
      | sbobj.Groups(5).Signals(4).YData = [0 0]
      | sbobj.Groups(5).TimeRange = [0 200]
  Z : Outport  VectorParamsAs1DForOutWhenUnconnected=off
  roll : Outport  Tag=STV Outport  Port=2  VectorParamsAs1DForOutWhenUnconnected=off
  pitch : Outport  Tag=STV Outport  Port=3  VectorParamsAs1DForOutWhenUnconnected=off
  Yaw : Outport  Tag=STV Outport  Port=4
  wires:
  Demux/4 -> Yaw/1
  Demux/3 -> pitch/1
  Demux/2 -> roll/1
  FromWs/1 -> Demux/1
  Demux/1 -> Z/1

== system three_a_attitude_control_euler/Commands/Roll ==
  Demux : Demux  Tag=STV Demux
      settings: DisplayOption=none
  FromWs : FromWorkspace  Tag=STV FromWs  VariableName=tuvar
      SigBuilderData=|
      | common.afterFinalStr = 'Extrapolate'
      | common.sampleTime = 0
      | dataSet(1).timeRange = [0 200]
      | dataSet(1).name = 'small_steps'
      | dataSet(2).timeRange = [0 200]
      | dataSet(2).name = 'zStairs_xyConstVEL'
      | dataSet(3).timeRange = [0 500]
      | dataSet(3).name = 'sineWaves'
      | dataSet(4).timeRange = [0 200]
      | dataSet(4).name = 'ZERO'
      | dataSet(5).timeRange = [0 200]
      | dataSet(5).name = 'SEARCH_P1'
      | sbobj.Name = 'Signal Builder'
      | sbobj.Groups(1).Name = 'small_steps'
      | sbobj.Groups(1).Signals(1).Name = 'Z'
      | sbobj.Groups(1).Signals(1).XData = [0 10 10.000001 20 20.000001 30 30.000001 55 200]
      | sbobj.Groups(1).Signals(1).YData = [0 0 2 2 2 2 2 2 2]
      | sbobj.Groups(1).Signals(2).Name = 'roll'
      | sbobj.Groups(1).Signals(2).XData = [0 10 10.000001 20 20.000001 30 30.000001 55 200]
      | sbobj.Groups(1).Signals(2).YData = [0 0 0 0 3 3 3 3 3]
      | sbobj.Groups(1).Signals(3).Name = 'pitch'
      | sbobj.Groups(1).Signals(3).XData = [0 10 10.000001 20 20.000001 30 30.000001 55 200]
      | sbobj.Groups(1).Signals(3).YData = [0 0 0 0 0 0 1 1 1]
      | sbobj.Groups(1).Signals(4).Name = 'Yaw'
      | sbobj.Groups(1).Signals(4).XData = [0 200]
      | sbobj.Groups(1).Signals(4).YData = [0 0]
      | sbobj.Groups(1).TimeRange = [0 200]
      | sbobj.Groups(2).Name = 'zStairs_xyConstVEL'
      | sbobj.Groups(2).Signals(1).Name = 'Z'
      | sbobj.Groups(2).Signals(1).XData = [0 10 10.000001 20 20.000001 30 30.000001 40 40.000001 55 200]
      | sbobj.Groups(2).Signals(1).YData = [0 0 1 1 2 2 1 1 0 0 0]
      | sbobj.Groups(2).Signals(2).Name = 'roll'
      | sbobj.Groups(2).Signals(2).XData = [0 10 10.000001 20 20.000001 30 30.000001 40 40.000001 55 200]
      | sbobj.Groups(2).Signals(2).YData = [0 1 1.0000001 2 2.0000001 3 3.0000001 4 4.0000001 5.5 20]
      | sbobj.Groups(2).Signals(3).Name = 'pitch'
      | sbobj.Groups(2).Signals(3).XData = [0 10 10.000001 20 20.000001 30 30.000001 40 40.000001 55 200]
      | sbobj.Groups(2).Signals(3).YData = [0 0.5 0.50000005 1 1.00000005 1.5 1.50000005 2 2.00000005 2.75 10]
      | sbobj.Groups(2).Signals(4).Name = 'Yaw'
      | sbobj.Groups(2).Signals(4).XData = [0 200]
      | sbobj.Groups(2).Signals(4).YData = [0 0]
      | sbobj.Groups(2).TimeRange = [0 200]
      | sbobj.Groups(3).Name = 'sineWaves'
      | sbobj.Groups(3).Signals(1).Name = 'Z'
      | sbobj.Groups(3).Signals(1).XData = [0 0.1 0.2 0.3 0.4 0.5 0.6 0.7 0.8 0.9 1 1.1 ... (5001 elements, 1x5001)]
      | sbobj.Groups(3).Signals(1).YData = [0 0.0314107325553 0.0627904665622 0.0941082340641 0.125333128258 0.156434333994 0.18738115819 0.218143060119 0.248689681547 0.278990876699 0.309016742004 0.338737645607 ... (5001 elements, 1x5001)]
      | sbobj.Groups(3).Signals(2).Name = 'roll'
      | sbobj.Groups(3).Signals(2).XData = [0 0.1 0.2 0.3 0.4 0.5 0.6 0.7 0.8 0.9 1 1.1 ... (5001 elements, 1x5001)]
      | sbobj.Groups(3).Signals(2).YData = [0 0.01 0.02 0.03 0.04 0.05 0.06 0.07 0.08 0.09 0.1 0.11 ... (5001 elements, 1x5001)]
      | sbobj.Groups(3).Signals(3).Name = 'pitch'
      | sbobj.Groups(3).Signals(3).XData = [0 0.1 0.2 0.3 0.4 0.5 0.6 0.7 0.8 0.9 1 1.1 ... (5001 elements, 1x5001)]
      | sbobj.Groups(3).Signals(3).YData = [0 0.0157073040455 0.0314107325553 0.04710641095 0.0627904665622 0.0784590295926 0.0941082340641 0.109734218776 0.125333128258 0.140901113717 0.156434333994 0.171928956505 ... (5001 elements, 1x5001)]
      | sbobj.Groups(3).Signals(4).Name = 'Yaw'
      | sbobj.Groups(3).Signals(4).XData = [0 500]
      | sbobj.Groups(3).Signals(4).YData = [0 0]
      | sbobj.Groups(3).TimeRange = [0 500]
      | sbobj.Groups(4).Name = 'ZERO'
      | sbobj.Groups(4).Signals(1).Name = 'Z'
      | sbobj.Groups(4).Signals(1).XData = [0 200]
      | sbobj.Groups(4).Signals(1).YData = [0 0]
      | sbobj.Groups(4).Signals(2).Name = 'roll'
      | sbobj.Groups(4).Signals(2).XData = [0 200]
      | sbobj.Groups(4).Signals(2).YData = [0 0]
      | sbobj.Groups(4).Signals(3).Name = 'pitch'
      | sbobj.Groups(4).Signals(3).XData = [0 200]
      | sbobj.Groups(4).Signals(3).YData = [0 0]
      | sbobj.Groups(4).Signals(4).Name = 'Yaw'
      | sbobj.Groups(4).Signals(4).XData = [0 200]
      | sbobj.Groups(4).Signals(4).YData = [0 0]
      | sbobj.Groups(4).TimeRange = [0 200]
      | sbobj.Groups(5).Name = 'SEARCH_P1'
      | sbobj.Groups(5).Signals(1).Name = 'Z'
      | sbobj.Groups(5).Signals(1).XData = [0 9.9 200]
      | sbobj.Groups(5).Signals(1).YData = [0 0 0]
      | sbobj.Groups(5).Signals(2).Name = 'roll'
      | sbobj.Groups(5).Signals(2).XData = [0 0.689655172414 1.37931034483 2.06896551724 2.75862068966 3.44827586207 4.13793103448 4.8275862069 5.51724137931 6.20689655172 6.89655172414 7.58620689655 ... (291 elements, 1x291)]
      | sbobj.Groups(5).Signals(2).YData = [0 5.37426100528 10.497227539 15.1293553798 19.0540513782 22.0878011112 24.088749813 24.9633353463 24.6706630635 23.2244179954 20.6922249539 17.1924864713 ... (291 elements, 1x291)]
      | sbobj.Groups(5).Signals(3).Name = 'pitch'
      | sbobj.Groups(5).Signals(3).XData = [0 200]
      | sbobj.Groups(5).Signals(3).YData = [0 0]
      | sbobj.Groups(5).Signals(4).Name = 'Yaw'
      | sbobj.Groups(5).Signals(4).XData = [0 200]
      | sbobj.Groups(5).Signals(4).YData = [0 0]
      | sbobj.Groups(5).TimeRange = [0 200]
  Z : Outport  VectorParamsAs1DForOutWhenUnconnected=off
  roll : Outport  Tag=STV Outport  Port=2  VectorParamsAs1DForOutWhenUnconnected=off
  pitch : Outport  Tag=STV Outport  Port=3  VectorParamsAs1DForOutWhenUnconnected=off
  Yaw : Outport  Tag=STV Outport  Port=4
  wires:
  Demux/4 -> Yaw/1
  Demux/3 -> pitch/1
  Demux/2 -> roll/1
  FromWs/1 -> Demux/1
  Demux/1 -> Z/1

== system three_a_attitude_control_euler/Commands/multisteps ==
  Demux : Demux  Tag=STV Demux
      settings: DisplayOption=none
  FromWs : FromWorkspace  Tag=STV FromWs  VariableName=tuvar
      SigBuilderData=|
      | common.afterFinalStr = 'Extrapolate'
      | common.sampleTime = 0
      | dataSet(1).timeRange = [0 200]
      | dataSet(1).name = 'small_steps'
      | dataSet(2).timeRange = [0 200]
      | dataSet(2).name = 'zStairs_xyConstVEL'
      | dataSet(3).timeRange = [0 500]
      | dataSet(3).name = 'sineWaves'
      | dataSet(4).timeRange = [0 200]
      | dataSet(4).name = 'ZERO'
      | dataSet(5).timeRange = [0 200]
      | dataSet(5).name = 'SEARCH_P1'
      | sbobj.Name = 'Signal Builder'
      | sbobj.Groups(1).Name = 'small_steps'
      | sbobj.Groups(1).Signals(1).Name = 'Z'
      | sbobj.Groups(1).Signals(1).XData = [0 10 10.000001 20 20.000001 30 30.000001 55 200]
      | sbobj.Groups(1).Signals(1).YData = [0 0 2 2 2 2 2 2 2]
      | sbobj.Groups(1).Signals(2).Name = 'roll'
      | sbobj.Groups(1).Signals(2).XData = [0 10 10.000001 20 20.000001 30 30.000001 55 200]
      | sbobj.Groups(1).Signals(2).YData = [0 0 0 0 3 3 3 3 3]
      | sbobj.Groups(1).Signals(3).Name = 'pitch'
      | sbobj.Groups(1).Signals(3).XData = [0 10 10.000001 20 20.000001 30 30.000001 55 200]
      | sbobj.Groups(1).Signals(3).YData = [0 0 0 0 0 0 1 1 1]
      | sbobj.Groups(1).Signals(4).Name = 'Yaw'
      | sbobj.Groups(1).Signals(4).XData = [0 200]
      | sbobj.Groups(1).Signals(4).YData = [0 0]
      | sbobj.Groups(1).TimeRange = [0 200]
      | sbobj.Groups(2).Name = 'zStairs_xyConstVEL'
      | sbobj.Groups(2).Signals(1).Name = 'Z'
      | sbobj.Groups(2).Signals(1).XData = [0 10 10.000001 20 20.000001 30 30.000001 40 40.000001 55 200]
      | sbobj.Groups(2).Signals(1).YData = [0 0 1 1 2 2 1 1 0 0 0]
      | sbobj.Groups(2).Signals(2).Name = 'roll'
      | sbobj.Groups(2).Signals(2).XData = [0 10 10.000001 20 20.000001 30 30.000001 40 40.000001 55 200]
      | sbobj.Groups(2).Signals(2).YData = [0 1 1.0000001 2 2.0000001 3 3.0000001 4 4.0000001 5.5 20]
      | sbobj.Groups(2).Signals(3).Name = 'pitch'
      | sbobj.Groups(2).Signals(3).XData = [0 10 10.000001 20 20.000001 30 30.000001 40 40.000001 55 200]
      | sbobj.Groups(2).Signals(3).YData = [0 0.5 0.50000005 1 1.00000005 1.5 1.50000005 2 2.00000005 2.75 10]
      | sbobj.Groups(2).Signals(4).Name = 'Yaw'
      | sbobj.Groups(2).Signals(4).XData = [0 200]
      | sbobj.Groups(2).Signals(4).YData = [0 0]
      | sbobj.Groups(2).TimeRange = [0 200]
      | sbobj.Groups(3).Name = 'sineWaves'
      | sbobj.Groups(3).Signals(1).Name = 'Z'
      | sbobj.Groups(3).Signals(1).XData = [0 0.1 0.2 0.3 0.4 0.5 0.6 0.7 0.8 0.9 1 1.1 ... (5001 elements, 1x5001)]
      | sbobj.Groups(3).Signals(1).YData = [0 0.0314107325553 0.0627904665622 0.0941082340641 0.125333128258 0.156434333994 0.18738115819 0.218143060119 0.248689681547 0.278990876699 0.309016742004 0.338737645607 ... (5001 elements, 1x5001)]
      | sbobj.Groups(3).Signals(2).Name = 'roll'
      | sbobj.Groups(3).Signals(2).XData = [0 0.1 0.2 0.3 0.4 0.5 0.6 0.7 0.8 0.9 1 1.1 ... (5001 elements, 1x5001)]
      | sbobj.Groups(3).Signals(2).YData = [0 0.01 0.02 0.03 0.04 0.05 0.06 0.07 0.08 0.09 0.1 0.11 ... (5001 elements, 1x5001)]
      | sbobj.Groups(3).Signals(3).Name = 'pitch'
      | sbobj.Groups(3).Signals(3).XData = [0 0.1 0.2 0.3 0.4 0.5 0.6 0.7 0.8 0.9 1 1.1 ... (5001 elements, 1x5001)]
      | sbobj.Groups(3).Signals(3).YData = [0 0.0157073040455 0.0314107325553 0.04710641095 0.0627904665622 0.0784590295926 0.0941082340641 0.109734218776 0.125333128258 0.140901113717 0.156434333994 0.171928956505 ... (5001 elements, 1x5001)]
      | sbobj.Groups(3).Signals(4).Name = 'Yaw'
      | sbobj.Groups(3).Signals(4).XData = [0 500]
      | sbobj.Groups(3).Signals(4).YData = [0 0]
      | sbobj.Groups(3).TimeRange = [0 500]
      | sbobj.Groups(4).Name = 'ZERO'
      | sbobj.Groups(4).Signals(1).Name = 'Z'
      | sbobj.Groups(4).Signals(1).XData = [0 200]
      | sbobj.Groups(4).Signals(1).YData = [0 0]
      | sbobj.Groups(4).Signals(2).Name = 'roll'
      | sbobj.Groups(4).Signals(2).XData = [0 200]
      | sbobj.Groups(4).Signals(2).YData = [0 0]
      | sbobj.Groups(4).Signals(3).Name = 'pitch'
      | sbobj.Groups(4).Signals(3).XData = [0 200]
      | sbobj.Groups(4).Signals(3).YData = [0 0]
      | sbobj.Groups(4).Signals(4).Name = 'Yaw'
      | sbobj.Groups(4).Signals(4).XData = [0 200]
      | sbobj.Groups(4).Signals(4).YData = [0 0]
      | sbobj.Groups(4).TimeRange = [0 200]
      | sbobj.Groups(5).Name = 'SEARCH_P1'
      | sbobj.Groups(5).Signals(1).Name = 'Z'
      | sbobj.Groups(5).Signals(1).XData = [0 7 27 32 52 57 77 82 102 107 127 132 157 187 200]
      | sbobj.Groups(5).Signals(1).YData = [0 5 5 5 5 5 5 5 5 5 5 5 5 0 0]
      | sbobj.Groups(5).Signals(2).Name = 'roll'
      | sbobj.Groups(5).Signals(2).XData = [0 7 27 32 52 57 77 82 102 107 127 132 157 187 200]
      | sbobj.Groups(5).Signals(2).YData = [0 5 25 25 5 5 25 25 5 5 25 25 0 0 0]
      | sbobj.Groups(5).Signals(3).Name = 'pitch'
      | sbobj.Groups(5).Signals(3).XData = [0 7 27 32 52 57 77 82 102 107 127 132 157 187 200]
      | sbobj.Groups(5).Signals(3).YData = [0 5 5 10 10 15 15 20 20 25 25 30 30 0 0]
      | sbobj.Groups(5).Signals(4).Name = 'Yaw'
      | sbobj.Groups(5).Signals(4).XData = [0 7 27 32 52 57 77 82 102 107 127 132 157 187 200]
      | sbobj.Groups(5).Signals(4).YData = [0 5 25 25 5 5 25 25 5 5 25 25 0 0 0]
      | sbobj.Groups(5).TimeRange = [0 200]
  Z : Outport  VectorParamsAs1DForOutWhenUnconnected=off
  roll : Outport  Tag=STV Outport  Port=2  VectorParamsAs1DForOutWhenUnconnected=off
  pitch : Outport  Tag=STV Outport  Port=3  VectorParamsAs1DForOutWhenUnconnected=off
  Yaw : Outport  Tag=STV Outport  Port=4
  wires:
  Demux/1 -> Z/1
  FromWs/1 -> Demux/1
  Demux/2 -> roll/1
  Demux/3 -> pitch/1
  Demux/4 -> Yaw/1

== system three_a_attitude_control_euler/Commands/yaw ==
  Demux : Demux  Tag=STV Demux
      settings: DisplayOption=none
  FromWs : FromWorkspace  Tag=STV FromWs  VariableName=tuvar
      SigBuilderData=|
      | common.afterFinalStr = 'Extrapolate'
      | common.sampleTime = 0
      | dataSet(1).timeRange = [0 200]
      | dataSet(1).name = 'small_steps'
      | dataSet(2).timeRange = [0 200]
      | dataSet(2).name = 'zStairs_xyConstVEL'
      | dataSet(3).timeRange = [0 500]
      | dataSet(3).name = 'sineWaves'
      | dataSet(4).timeRange = [0 200]
      | dataSet(4).name = 'ZERO'
      | dataSet(5).timeRange = [0 200]
      | dataSet(5).name = 'SEARCH_P1'
      | sbobj.Name = 'Signal Builder'
      | sbobj.Groups(1).Name = 'small_steps'
      | sbobj.Groups(1).Signals(1).Name = 'Z'
      | sbobj.Groups(1).Signals(1).XData = [0 10 10.000001 20 20.000001 30 30.000001 55 200]
      | sbobj.Groups(1).Signals(1).YData = [0 0 2 2 2 2 2 2 2]
      | sbobj.Groups(1).Signals(2).Name = 'roll'
      | sbobj.Groups(1).Signals(2).XData = [0 10 10.000001 20 20.000001 30 30.000001 55 200]
      | sbobj.Groups(1).Signals(2).YData = [0 0 0 0 3 3 3 3 3]
      | sbobj.Groups(1).Signals(3).Name = 'pitch'
      | sbobj.Groups(1).Signals(3).XData = [0 10 10.000001 20 20.000001 30 30.000001 55 200]
      | sbobj.Groups(1).Signals(3).YData = [0 0 0 0 0 0 1 1 1]
      | sbobj.Groups(1).Signals(4).Name = 'Yaw'
      | sbobj.Groups(1).Signals(4).XData = [0 200]
      | sbobj.Groups(1).Signals(4).YData = [0 0]
      | sbobj.Groups(1).TimeRange = [0 200]
      | sbobj.Groups(2).Name = 'zStairs_xyConstVEL'
      | sbobj.Groups(2).Signals(1).Name = 'Z'
      | sbobj.Groups(2).Signals(1).XData = [0 10 10.000001 20 20.000001 30 30.000001 40 40.000001 55 200]
      | sbobj.Groups(2).Signals(1).YData = [0 0 1 1 2 2 1 1 0 0 0]
      | sbobj.Groups(2).Signals(2).Name = 'roll'
      | sbobj.Groups(2).Signals(2).XData = [0 10 10.000001 20 20.000001 30 30.000001 40 40.000001 55 200]
      | sbobj.Groups(2).Signals(2).YData = [0 1 1.0000001 2 2.0000001 3 3.0000001 4 4.0000001 5.5 20]
      | sbobj.Groups(2).Signals(3).Name = 'pitch'
      | sbobj.Groups(2).Signals(3).XData = [0 10 10.000001 20 20.000001 30 30.000001 40 40.000001 55 200]
      | sbobj.Groups(2).Signals(3).YData = [0 0.5 0.50000005 1 1.00000005 1.5 1.50000005 2 2.00000005 2.75 10]
      | sbobj.Groups(2).Signals(4).Name = 'Yaw'
      | sbobj.Groups(2).Signals(4).XData = [0 200]
      | sbobj.Groups(2).Signals(4).YData = [0 0]
      | sbobj.Groups(2).TimeRange = [0 200]
      | sbobj.Groups(3).Name = 'sineWaves'
      | sbobj.Groups(3).Signals(1).Name = 'Z'
      | sbobj.Groups(3).Signals(1).XData = [0 0.1 0.2 0.3 0.4 0.5 0.6 0.7 0.8 0.9 1 1.1 ... (5001 elements, 1x5001)]
      | sbobj.Groups(3).Signals(1).YData = [0 0.0314107325553 0.0627904665622 0.0941082340641 0.125333128258 0.156434333994 0.18738115819 0.218143060119 0.248689681547 0.278990876699 0.309016742004 0.338737645607 ... (5001 elements, 1x5001)]
      | sbobj.Groups(3).Signals(2).Name = 'roll'
      | sbobj.Groups(3).Signals(2).XData = [0 0.1 0.2 0.3 0.4 0.5 0.6 0.7 0.8 0.9 1 1.1 ... (5001 elements, 1x5001)]
      | sbobj.Groups(3).Signals(2).YData = [0 0.01 0.02 0.03 0.04 0.05 0.06 0.07 0.08 0.09 0.1 0.11 ... (5001 elements, 1x5001)]
      | sbobj.Groups(3).Signals(3).Name = 'pitch'
      | sbobj.Groups(3).Signals(3).XData = [0 0.1 0.2 0.3 0.4 0.5 0.6 0.7 0.8 0.9 1 1.1 ... (5001 elements, 1x5001)]
      | sbobj.Groups(3).Signals(3).YData = [0 0.0157073040455 0.0314107325553 0.04710641095 0.0627904665622 0.0784590295926 0.0941082340641 0.109734218776 0.125333128258 0.140901113717 0.156434333994 0.171928956505 ... (5001 elements, 1x5001)]
      | sbobj.Groups(3).Signals(4).Name = 'Yaw'
      | sbobj.Groups(3).Signals(4).XData = [0 500]
      | sbobj.Groups(3).Signals(4).YData = [0 0]
      | sbobj.Groups(3).TimeRange = [0 500]
      | sbobj.Groups(4).Name = 'ZERO'
      | sbobj.Groups(4).Signals(1).Name = 'Z'
      | sbobj.Groups(4).Signals(1).XData = [0 200]
      | sbobj.Groups(4).Signals(1).YData = [0 0]
      | sbobj.Groups(4).Signals(2).Name = 'roll'
      | sbobj.Groups(4).Signals(2).XData = [0 200]
      | sbobj.Groups(4).Signals(2).YData = [0 0]
      | sbobj.Groups(4).Signals(3).Name = 'pitch'
      | sbobj.Groups(4).Signals(3).XData = [0 200]
      | sbobj.Groups(4).Signals(3).YData = [0 0]
      | sbobj.Groups(4).Signals(4).Name = 'Yaw'
      | sbobj.Groups(4).Signals(4).XData = [0 200]
      | sbobj.Groups(4).Signals(4).YData = [0 0]
      | sbobj.Groups(4).TimeRange = [0 200]
      | sbobj.Groups(5).Name = 'SEARCH_P1'
      | sbobj.Groups(5).Signals(1).Name = 'Z'
      | sbobj.Groups(5).Signals(1).XData = [0 9.9 200]
      | sbobj.Groups(5).Signals(1).YData = [0 0 0]
      | sbobj.Groups(5).Signals(2).Name = 'roll'
      | sbobj.Groups(5).Signals(2).XData = [0 200]
      | sbobj.Groups(5).Signals(2).YData = [0 0]
      | sbobj.Groups(5).Signals(3).Name = 'pitch'
      | sbobj.Groups(5).Signals(3).XData = [0 200]
      | sbobj.Groups(5).Signals(3).YData = [0 0]
      | sbobj.Groups(5).Signals(4).Name = 'Yaw'
      | sbobj.Groups(5).Signals(4).XData = [0 1.05263157895 2.10526315789 3.15789473684 4.21052631579 5.26315789474 6.31578947368 7.36842105263 8.42105263158 9.47368421053 10.5263157895 11.5789473684 ... (191 elements, 1x191)]
      | sbobj.Groups(5).Signals(4).YData = [0 22.7289628443 42.9948898883 58.6016534784 67.8580186158 69.7609145105 64.1041328659 51.5006737471 33.3163175126 11.5216213197 -11.5216213197 -33.3163175126 ... (191 elements, 1x191)]
      | sbobj.Groups(5).TimeRange = [0 200]
  Z : Outport  VectorParamsAs1DForOutWhenUnconnected=off
  roll : Outport  Tag=STV Outport  Port=2  VectorParamsAs1DForOutWhenUnconnected=off
  pitch : Outport  Tag=STV Outport  Port=3  VectorParamsAs1DForOutWhenUnconnected=off
  Yaw : Outport  Tag=STV Outport  Port=4
  wires:
  Demux/4 -> Yaw/1
  Demux/3 -> pitch/1
  Demux/2 -> roll/1
  FromWs/1 -> Demux/1
  Demux/1 -> Z/1

== system three_a_attitude_control_euler/Control allocation and motor control/Ideal Actuators with allocation ==
  THRUST_CMD : Inport
  TQ_Roll_CMD : Inport  Port=2
  TQ_Pitch_CMD : Inport  Port=3
  TQ_Yaw_CMD : Inport  Port=4
  Control allocation : Subsystem
  Perfect actuators : Subsystem  VariantControl=Choice2
  Thrust : Outport
  Mx : Outport  Port=2
  My : Outport  Port=3
  Mz : Outport  Port=4
  T_actual : Outport  Port=5
  w_mot_actual : Outport  Port=6
  wires:
  Control allocation/1(w_command) -> Perfect actuators/1(w_cmd)
  THRUST_CMD/1 -> Control allocation/1(THRUST_CMD)
  TQ_Pitch_CMD/1 -> Control allocation/3(TQ_Pitch_CMD)
  TQ_Roll_CMD/1 -> Control allocation/2(TQ_Roll_CMD)
  TQ_Yaw_CMD/1 -> Control allocation/4(TQ_Yaw_CMD)
  Perfect actuators/5(T_actual) -> T_actual/1
  Perfect actuators/6(w_mot_actual) -> w_mot_actual/1
  Perfect actuators/3(My) -> My/1
  Perfect actuators/2(Mx) -> Mx/1
  Perfect actuators/4(Mz) -> Mz/1
  Perfect actuators/1(Thrust) -> Thrust/1

== system three_a_attitude_control_euler/Control allocation and motor control/Ideal Actuattion (direct transfer) ==
  THRUST_CMD : Inport
  TQ_Roll_CMD : Inport  Port=2
  TQ_Pitch_CMD : Inport  Port=3
  TQ_Yaw_CMD : Inport  Port=4
  Mux : Mux
  Zero : Constant  Value=[0;0;0;0]  OutDataTypeStr=Inherit: Inherit via back propagation
  Thrust : Outport
  Mx : Outport  Port=2
  My : Outport  Port=3
  Mz : Outport  Port=4
  T_actual : Outport  Port=5
  w_mot_actual : Outport  Port=6
  wires:
  Zero/1 -> w_mot_actual/1
  TQ_Pitch_CMD/1 -> Mux/3, My/1
  TQ_Roll_CMD/1 -> Mux/2, Mx/1
  TQ_Yaw_CMD/1 -> Mux/4, Mz/1
  THRUST_CMD/1 -> Mux/1, Thrust/1
  Mux/1 -> T_actual/1

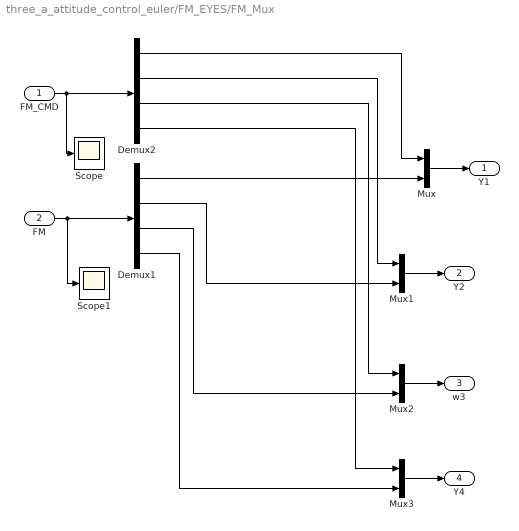
== system three_a_attitude_control_euler/FM_EYES/FM_Mux ==
  FM_CMD : Inport
  FM : Inport  Port=2
  Demux1 : Demux
  Demux2 : Demux
  Mux{,1..3} (4 alike) : Mux  Inputs=2
  Scope : Scope
  Scope1 : Scope
  Y1 : Outport  VectorParamsAs1DForOutWhenUnconnected=off
  Y2 : Outport  Port=2  VectorParamsAs1DForOutWhenUnconnected=off
  w3 : Outport  Port=3  VectorParamsAs1DForOutWhenUnconnected=off
  Y4 : Outport  Port=4  VectorParamsAs1DForOutWhenUnconnected=off
  wires:
  FM_CMD/1 -> Scope/1, Demux2/1
  FM/1 -> Scope1/1, Demux1/1
  Mux/1 -> Y1/1
  Mux1/1 -> Y2/1
  Mux3/1 -> Y4/1
  Mux2/1 -> w3/1
  Demux2/1 -> Mux/1
  Demux2/2 -> Mux1/1
  Demux2/3 -> Mux2/1
  Demux2/4 -> Mux3/1
  Demux1/1 -> Mux/2
  Demux1/2 -> Mux1/2
  Demux1/3 -> Mux2/2
  Demux1/4 -> Mux3/2

== system three_a_attitude_control_euler/Quad_EOM/Calc DCM ==
  Euler angs : Inport
  Calculate DCM bRw : MATLAB Function  TreatAsAtomicUnit=on
  Demux3 : Demux  Outputs=3
  bRg : Outport
  wires:
  Calculate DCM bRw/1(bRw) -> bRg/1
  Demux3/2 -> Calculate DCM bRw/2(theta_t)  "thetsa"
  Demux3/3 -> Calculate DCM bRw/3(psi_t)  "psi"
  Demux3/1 -> Calculate DCM bRw/1(phi_t)  "phi"
  Euler angs/1 -> Demux3/1

== system three_a_attitude_control_euler/Quad_EOM/Calc Euler_rates ==
  "p q r " : Inport
  Euler_angs : Inport  Port=2
  Demux1 : Demux  Outputs=3
  Demux2 : Demux  Outputs=3
  Demux3 : Demux  Outputs=3
  Mux1 : Mux  Inputs=3
  Reshape1 : Reshape  OutputDimensionality=Column vector (2-D)
  Reshape2 : Reshape  OutputDimensionality=Column vector (2-D)
  Terminator : Terminator
  euler_rates : MATLAB Function  TreatAsAtomicUnit=on
  Euler_rates : Outport
  wires:
  Demux2/2 -> Mux1/2  "thetadot_Y2_pitch"
  Demux1/1 -> euler_rates/1(phi_t)  "phi"
  Demux3/2 -> euler_rates/4(q)
  Demux2/1 -> Mux1/1  "phidot_Z1_yaw"
  "p q r "/1 -> Reshape1/1
  Euler_angs/1 -> Demux1/1
  Demux3/1 -> euler_rates/3(p)
  Reshape2/1 -> Euler_rates/1
  Reshape1/1 -> Demux3/1  "wb"
  Demux3/3 -> euler_rates/5(r)
  Demux1/3 -> Terminator/1  "psi"
  euler_rates/1(euler_rates) -> Demux2/1  "euler_rates"
  Demux1/2 -> euler_rates/2(theta_t)  "theta"
  Mux1/1 -> Reshape2/1
  Demux2/3 -> Mux1/3  "psidot_X3_roll"

== system three_a_attitude_control_euler/Quad_EOM/Gravity_G_to_B ==
  note: F_B = ^BR_G * F_G
  bRg : Inport
  Product : Product  Multiplication=Matrix(*)
  Product1 : Product
  gravity vector in inertial frame : Constant  Value=[0;0;g]  VectorParams1D=off
  mass : Constant  Value=m
  Fb_gravity : Outport  VectorParamsAs1DForOutWhenUnconnected=off
  wires:
  bRg/1 -> Product/1
  Product/1 -> Fb_gravity/1  "F_garvity in body frame"
  Product1/1 -> Product/2  "m*g"
  gravity vector in inertial frame/1 -> Product1/1  "Fg"
  mass/1 -> Product1/2
